simulink model "ElevatorPlant_Storage_A"  (R2015b)
settings: Solver=VariableStepAuto  StartTime=0.0  StopTime=10.0  RelTol=1e-3
(part 2 of 8)

== stateflow chart ElevatorPlant_Storage_A/Elevator Plant_storage ==
  state Init_procedure
    state BLK_Init
      %BLK(LPS0)
      %BLK(LPD1)
      %BLK(LPS1)
      %BLK(LPD2)
      %BLK(LPS2)
      %BLK(LPD3)
    state Closing_all_doors
      state Closing0
        state Reset
          state Reset_0
            en:
            LPS0=false;
            BUTTON_CAR(1)=false;
            BUTTON_UP(1)=false;
          state Reset_1
            en:
            LPS1=false;
            LPD1=false;
            BUTTON_CAR(2)=false;
            BUTTON_UP(2)=false;
            BUTTON_DOWN(2)=false;
          state Reset_2
            en:
            LPS2=false;
            LPD2=false;
            BUTTON_CAR(3)=false;
            BUTTON_UP(3)=false;
            BUTTON_DOWN(3)=false;
          state Reset_3
            en:
            LPD3=false;
            BUTTON_CAR(4)=false;
            BUTTON_DOWN(4)=false;
          (default) -> (junction 27093)
          (junction 27093) -> Init_procedure.Closing_all_doors.Closing0.Reset.Reset_0 [order 1] : [FLOOR==0]
          Init_procedure.Closing_all_doors.Closing0.Reset.Reset_0 -> (junction 27101)
          (junction 27093) -> (junction 27095) [order 2]
          (junction 27101) -> (junction 27103)
          (junction 27095) -> Init_procedure.Closing_all_doors.Closing0.Reset.Reset_1 [order 1] : [FLOOR==1]
          Init_procedure.Closing_all_doors.Closing0.Reset.Reset_1 -> (junction 27103)
          (junction 27095) -> (junction 27097) [order 2]
          (junction 27103) -> (junction 27104)
          (junction 27097) -> Init_procedure.Closing_all_doors.Closing0.Reset.Reset_2 [order 1] : [FLOOR==2]
          Init_procedure.Closing_all_doors.Closing0.Reset.Reset_2 -> (junction 27104)
          (junction 27097) -> (junction 27099) [order 2]
          (junction 27104) -> (junction 27109)
          (junction 27099) -> Init_procedure.Closing_all_doors.Closing0.Reset.Reset_3 [order 1] : [FLOOR==3]
          Init_procedure.Closing_all_doors.Closing0.Reset.Reset_3 -> (junction 27109)
          (junction 27099) -> (junction 27114) [order 2]
          (junction 27109) -> (junction 27115)
          (junction 27115) -> (junction 27114)
        state Timer_close
          state Set_tmr
            en: Q_cl=true;
          state Set
            en:PT_cl=5;
            IN_cl=true;
          state Counting
            en:ET_cl = ET_cl + 1;
            Q_cl=false;
          (junction 11293) -> Init_procedure.Closing_all_doors.Closing0.Timer_close.Set_tmr [order 1] : [ET_cl==PT_cl]
          Init_procedure.Closing_all_doors.Closing0.Timer_close.Set_tmr -> (junction 11294)
          (default) -> Init_procedure.Closing_all_doors.Closing0.Timer_close.Set
          Init_procedure.Closing_all_doors.Closing0.Timer_close.Counting -> (junction 11293)
          (junction 11293) -> (junction 11294) [order 2]
          Init_procedure.Closing_all_doors.Closing0.Timer_close.Set -> (junction 11295)
          (junction 11295) -> Init_procedure.Closing_all_doors.Closing0.Timer_close.Counting [order 1] : [ET_cl<PT_cl]
          (junction 11295) -> (junction 11294) [order 2]
        state Closing
          en: CP0=Q_cl;
        state Button_detection
          state Save_energy
            en:
            LL=not(Q_LL);
          state Timer_LL
            state Set_tmr
              en:
              Q_LL=true;
            state Counting
              en:
              ET_LL= ET_LL + 1;
              Q_LL=false;
            state Set
              en:
              IN_LL=true;
              PT_LL=10;
            (junction 66372) -> Init_procedure.Closing_all_doors.Closing0.Button_detection.Timer_LL.Set_tmr [order 1] : [ET_LL==PT_LL]
            Init_procedure.Closing_all_doors.Closing0.Button_detection.Timer_LL.Set_tmr -> (junction 66373)
            Init_procedure.Closing_all_doors.Closing0.Button_detection.Timer_LL.Counting -> (junction 66372)
            (junction 66372) -> (junction 66373) [order 2]
            (default) -> Init_procedure.Closing_all_doors.Closing0.Button_detection.Timer_LL.Set
            Init_procedure.Closing_all_doors.Closing0.Button_detection.Timer_LL.Set -> (junction 66374)
            (junction 66374) -> Init_procedure.Closing_all_doors.Closing0.Button_detection.Timer_LL.Counting [order 1] : [ET_LL<PT_LL]
            (junction 66374) -> (junction 66373) [order 2]
          state BUTTON_DOWN
            state Button_DOWN_1
              en:
              BUTTON_DOWN(2)=true;
              BUT_TEMP=1;
              LPD1=true;
              PUSHED=true;
              UPDATE=false;
              IN_LL=false; ET_LL=0;
            state First_but_1
              en:
              BUT_1=BUT_TEMP;
              FIRST_BUT=false;
            state Button_DOWN_2
              en:
              BUTTON_DOWN(3)=true;
              BUT_TEMP=2;
              LPD2=true;
              PUSHED=true;
              UPDATE=false;
              IN_LL=false; ET_LL=0;
            state First_but_2
              en:
              BUT_1=BUT_TEMP;
              FIRST_BUT=false;
            state Button_DOWN_3
              en:
              BUTTON_DOWN(4)=true;
              BUT_TEMP=3;
              LPD3=true;
              PUSHED=true;
              UPDATE=false;
              IN_LL=false; ET_LL=0;
            state First_but_3
              en:
              BUT_1=BUT_TEMP;
              FIRST_BUT=false;
            (default) -> (junction 66387)
            (junction 66387) -> Init_procedure.Closing_all_doors.Closing0.Button_detection.BUTTON_DOWN.Button_DOWN_1 [order 1] : [PD1]
            Init_procedure.Closing_all_doors.Closing0.Button_detection.BUTTON_DOWN.Button_DOWN_1 -> (junction 66388)
            (junction 66388) -> Init_procedure.Closing_all_doors.Closing0.Button_detection.BUTTON_DOWN.First_but_1 [order 1] : [FIRST_BUT && not(RPC1)]
            Init_procedure.Closing_all_doors.Closing0.Button_detection.BUTTON_DOWN.First_but_1 -> (junction 66389)
            (junction 66387) -> (junction 66390) [order 2]
            (junction 66388) -> (junction 66391) [order 2]
            (junction 66389) -> (junction 66392)
            (junction 66391) -> (junction 66390)
            (junction 66392) -> (junction 66391)
            (junction 66390) -> (junction 66393)
            (junction 66393) -> Init_procedure.Closing_all_doors.Closing0.Button_detection.BUTTON_DOWN.Button_DOWN_2 [order 1] : [PD2]
            Init_procedure.Closing_all_doors.Closing0.Button_detection.BUTTON_DOWN.Button_DOWN_2 -> (junction 66394)
            (junction 66394) -> Init_procedure.Closing_all_doors.Closing0.Button_detection.BUTTON_DOWN.First_but_2 [order 1] : [FIRST_BUT && not(RPC2)]
            Init_procedure.Closing_all_doors.Closing0.Button_detection.BUTTON_DOWN.First_but_2 -> (junction 66395)
            (junction 66393) -> (junction 66396) [order 2]
            (junction 66394) -> (junction 66397) [order 2]
            (junction 66395) -> (junction 66398)
            (junction 66397) -> (junction 66396)
            (junction 66398) -> (junction 66397)
            (junction 66396) -> (junction 66399)
            (junction 66399) -> Init_procedure.Closing_all_doors.Closing0.Button_detection.BUTTON_DOWN.Button_DOWN_3 [order 1] : [PD3]
            Init_procedure.Closing_all_doors.Closing0.Button_detection.BUTTON_DOWN.Button_DOWN_3 -> (junction 66400)
            (junction 66400) -> Init_procedure.Closing_all_doors.Closing0.Button_detection.BUTTON_DOWN.First_but_3 [order 1] : [FIRST_BUT && not(RPC3)]
            Init_procedure.Closing_all_doors.Closing0.Button_detection.BUTTON_DOWN.First_but_3 -> (junction 66401)
            (junction 66399) -> (junction 66402) [order 2]
            (junction 66400) -> (junction 66403) [order 2]
            (junction 66401) -> (junction 66404)
            (junction 66403) -> (junction 66402)
            (junction 66404) -> (junction 66403)
          state BUTTON_CAR
            state Button_CAR_0
              en:
              BUTTON_CAR(1)=true;
              BUT_TEMP=0;
              LPC0=true;
              PUSHED=true;
              UPDATE=false;
              IN_LL=false; ET_LL=0;
            state First_but_0
              en:
              BUT_1=BUT_TEMP;
              FIRST_BUT=false;
            state Button_CAR_1
              en:
              BUTTON_CAR(2)=true;
              BUT_TEMP=1;
              LPC1=true;
              PUSHED=true;
              UPDATE=false;
              IN_LL=false; ET_LL=0;
            state First_but_1
              en:
              BUT_1=BUT_TEMP;
              FIRST_BUT=false;
            state Button_CAR_2
              en:
              BUTTON_CAR(3)=true;
              BUT_TEMP=2;
              LPC2=true;
              PUSHED=true;
              UPDATE=false;
              IN_LL=false; ET_LL=0;
            state First_but_2
              en:
              BUT_1=BUT_TEMP;
              FIRST_BUT=false;
            state Button_CAR_3
              en:
              BUTTON_CAR(4)=true;
              BUT_TEMP=3;
              LPC3=true;
              PUSHED=true;
              UPDATE=false;
              IN_LL=false; ET_LL=0;
            state First_but_3
              en:
              BUT_1=BUT_TEMP;
              FIRST_BUT=false;
            (default) -> (junction 66442)
            (junction 66442) -> Init_procedure.Closing_all_doors.Closing0.Button_detection.BUTTON_CAR.Button_CAR_0 [order 1] : [P0]
            Init_procedure.Closing_all_doors.Closing0.Button_detection.BUTTON_CAR.Button_CAR_0 -> (junction 66443)
            (junction 66443) -> Init_procedure.Closing_all_doors.Closing0.Button_detection.BUTTON_CAR.First_but_0 [order 1] : [FIRST_BUT && not(RPC0)]
            Init_procedure.Closing_all_doors.Closing0.Button_detection.BUTTON_CAR.First_but_0 -> (junction 66444)
            (junction 66442) -> (junction 66445) [order 2]
            (junction 66443) -> (junction 66446) [order 2]
            (junction 66444) -> (junction 66447)
            (junction 66446) -> (junction 66445)
            (junction 66447) -> (junction 66446)
            (junction 66445) -> (junction 66450)
            Init_procedure.Closing_all_doors.Closing0.Button_detection.BUTTON_CAR.Button_CAR_1 -> (junction 66448)
            (junction 66448) -> Init_procedure.Closing_all_doors.Closing0.Button_detection.BUTTON_CAR.First_but_1 [order 1] : [FIRST_BUT && not(RPC1)]
            Init_procedure.Closing_all_doors.Closing0.Button_detection.BUTTON_CAR.First_but_1 -> (junction 66449)
            (junction 66448) -> (junction 66452) [order 2]
            (junction 66449) -> (junction 66453)
            (junction 66450) -> Init_procedure.Closing_all_doors.Closing0.Button_detection.BUTTON_CAR.Button_CAR_1 [order 1] : [P1]
            (junction 66450) -> (junction 66451) [order 2]
            (junction 66452) -> (junction 66451)
            (junction 66453) -> (junction 66452)
            (junction 66451) -> (junction 66454)
            (junction 66454) -> Init_procedure.Closing_all_doors.Closing0.Button_detection.BUTTON_CAR.Button_CAR_2 [order 1] : [P2]
            Init_procedure.Closing_all_doors.Closing0.Button_detection.BUTTON_CAR.Button_CAR_2 -> (junction 66455)
            (junction 66455) -> Init_procedure.Closing_all_doors.Closing0.Button_detection.BUTTON_CAR.First_but_2 [order 1] : [FIRST_BUT && not(RPC2)]
            Init_procedure.Closing_all_doors.Closing0.Button_detection.BUTTON_CAR.First_but_2 -> (junction 66456)
            (junction 66454) -> (junction 66457) [order 2]
            (junction 66455) -> (junction 66458) [order 2]
            (junction 66456) -> (junction 66459)
            (junction 66458) -> (junction 66457)
            (junction 66459) -> (junction 66458)
            (junction 66457) -> (junction 66460)
            (junction 66460) -> Init_procedure.Closing_all_doors.Closing0.Button_detection.BUTTON_CAR.Button_CAR_3 [order 1] : [P3]
            Init_procedure.Closing_all_doors.Closing0.Button_detection.BUTTON_CAR.Button_CAR_3 -> (junction 66461)
            (junction 66461) -> Init_procedure.Closing_all_doors.Closing0.Button_detection.BUTTON_CAR.First_but_3 [order 1] : [FIRST_BUT && not(RPC3)]
            Init_procedure.Closing_all_doors.Closing0.Button_detection.BUTTON_CAR.First_but_3 -> (junction 66462)
            (junction 66460) -> (junction 66463) [order 2]
            (junction 66461) -> (junction 66464) [order 2]
            (junction 66462) -> (junction 66465)
            (junction 66464) -> (junction 66463)
            (junction 66465) -> (junction 66464)
          state BUTTON_UP
            state Button_UP_0
              en:
              BUTTON_UP(1)=true;
              BUT_TEMP=0;
              LPS0=true;
              PUSHED=true;
              UPDATE=false;
              IN_LL=false; ET_LL=0;
            state First_but_0
              en:
              BUT_1=BUT_TEMP;
              FIRST_BUT=false;
            state Button_UP_1
              en:
              BUTTON_UP(2)=true;
              BUT_TEMP=1;
              LPS1=true;
              PUSHED=true;
              UPDATE=false;
              IN_LL=false; ET_LL=0;
            state First_but_1
              en:
              BUT_1=BUT_TEMP;
              FIRST_BUT=false;
            state Button_UP_2
              en:
              BUTTON_UP(3)=true;
              BUT_TEMP=2;
              LPS2=true;
              PUSHED=true;
              UPDATE=false;
              IN_LL=false; ET_LL=0;
            state First_but_2
              en:
              BUT_1=BUT_TEMP;
              FIRST_BUT=false;
            (junction 66515) -> Init_procedure.Closing_all_doors.Closing0.Button_detection.BUTTON_UP.Button_UP_0 [order 1] : [PS0]
            Init_procedure.Closing_all_doors.Closing0.Button_detection.BUTTON_UP.Button_UP_0 -> (junction 66516)
            (junction 66516) -> Init_procedure.Closing_all_doors.Closing0.Button_detection.BUTTON_UP.First_but_0 [order 1] : [FIRST_BUT && not(RPC0)]
            Init_procedure.Closing_all_doors.Closing0.Button_detection.BUTTON_UP.First_but_0 -> (junction 66517)
            (default) -> (junction 66515)
            (junction 66515) -> (junction 66520) [order 2]
            (junction 66516) -> (junction 66518) [order 2]
            (junction 66517) -> (junction 66519)
            (junction 66519) -> (junction 66518)
            (junction 66518) -> (junction 66520)
            (junction 66520) -> (junction 66521)
            (junction 66521) -> Init_procedure.Closing_all_doors.Closing0.Button_detection.BUTTON_UP.Button_UP_1 [order 1] : [PS1]
            Init_procedure.Closing_all_doors.Closing0.Button_detection.BUTTON_UP.Button_UP_1 -> (junction 66522)
            (junction 66522) -> Init_procedure.Closing_all_doors.Closing0.Button_detection.BUTTON_UP.First_but_1 [order 1] : [FIRST_BUT && not(RPC1)]
            Init_procedure.Closing_all_doors.Closing0.Button_detection.BUTTON_UP.First_but_1 -> (junction 66523)
            (junction 66521) -> (junction 66524) [order 2]
            (junction 66522) -> (junction 66525) [order 2]
            (junction 66523) -> (junction 66526)
            (junction 66525) -> (junction 66524)
            (junction 66526) -> (junction 66525)
            (junction 66524) -> (junction 66528)
            Init_procedure.Closing_all_doors.Closing0.Button_detection.BUTTON_UP.First_but_2 -> (junction 66527)
            (junction 66527) -> (junction 66532)
            (junction 66528) -> Init_procedure.Closing_all_doors.Closing0.Button_detection.BUTTON_UP.Button_UP_2 [order 1] : [PS2]
            Init_procedure.Closing_all_doors.Closing0.Button_detection.BUTTON_UP.Button_UP_2 -> (junction 66529)
            (junction 66529) -> Init_procedure.Closing_all_doors.Closing0.Button_detection.BUTTON_UP.First_but_2 [order 1] : [FIRST_BUT && not(RPC2)]
            (junction 66528) -> (junction 66530) [order 2]
            (junction 66529) -> (junction 66531) [order 2]
            (junction 66531) -> (junction 66530)
            (junction 66532) -> (junction 66531)
          state Max_Min_assignment
            state Min_but
              en:
              BUTTON=MIN_BUT;
            state Max_but
              en:
              BUTTON=MAX_BUT;
            state First_but
              en:
              BUTTON=BUT_1;
            state Max_but1
              en:
              MAX_BUT=2;
            state Max_but2
              en:
              MAX_BUT=1;
            state Max_but3
              en:
              MAX_BUT=0;
            state Min_but1
              en:
              MIN_BUT=1;
            state Min_but2
              en:
              MIN_BUT=2;
            state Min_but3
              en:
              MIN_BUT=3;
            state MAX
              en:
              MAX_BUT=BUT_TEMP;
            state MIN
              en:
              MIN_BUT=BUT_TEMP;
            state Updating_button_0
              en:
              BUTTON=MAX_BUT;
            state Updating_button_1
              en:
              BUTTON=MIN_BUT;
            (junction 66570) -> Init_procedure.Closing_all_doors.Closing0.Button_detection.Max_Min_assignment.Min_but [order 1] : [(MAX_BUT-FLOOR)>(FLOOR-MIN_BUT)]
            Init_procedure.Closing_all_doors.Closing0.Button_detection.Max_Min_assignment.Min_but -> (junction 66571)
            (junction 66572) -> (junction 66570) [order 1] : [not(FLAG_STOP) && MOTION==2 && FLAG==3]
            (default) -> (junction 66572)
            (junction 66570) -> (junction 66573) [order 2]
            (junction 66571) -> (junction 66574)
            (junction 66572) -> (junction 66575) [order 2]
            (junction 66573) -> Init_procedure.Closing_all_doors.Closing0.Button_detection.Max_Min_assignment.Max_but [order 1] : [(MAX_BUT-FLOOR)<(FLOOR-MIN_BUT)]
            Init_procedure.Closing_all_doors.Closing0.Button_detection.Max_Min_assignment.Max_but -> (junction 66574)
            (junction 66573) -> Init_procedure.Closing_all_doors.Closing0.Button_detection.Max_Min_assignment.First_but [order 2]
            (junction 66574) -> (junction 66577)
            Init_procedure.Closing_all_doors.Closing0.Button_detection.Max_Min_assignment.First_but -> (junction 66576)
            (junction 66576) -> (junction 66575)
            (junction 66577) -> (junction 66576)
            (junction 66575) -> (junction 66578)
            (junction 66579) -> (junction 66580) [order 1] : [MOTION==0]
                | {MOTION=1;
                | UPDATE=true;}
            (junction 66580) -> Init_procedure.Closing_all_doors.Closing0.Button_detection.Max_Min_assignment.Max_but1 [order 1] : [BUTTON_UP(2)]
            Init_procedure.Closing_all_doors.Closing0.Button_detection.Max_Min_assignment.Max_but1 -> (junction 66581)
            (junction 66578) -> (junction 66579) [order 1] : [BUTTON==FLOOR && EXTEND]
                | {EXTEND=false;}
            (junction 66578) -> (junction 66592) [order 2]
            (junction 66579) -> (junction 66584) [order 2]
            (junction 66580) -> (junction 66582) [order 2]
            (junction 66581) -> (junction 66583)
            (junction 66582) -> Init_procedure.Closing_all_doors.Closing0.Button_detection.Max_Min_assignment.Max_but2 [order 1] : [BUTTON_UP(1)]
            Init_procedure.Closing_all_doors.Closing0.Button_detection.Max_Min_assignment.Max_but2 -> (junction 66583)
            (junction 66582) -> Init_procedure.Closing_all_doors.Closing0.Button_detection.Max_Min_assignment.Max_but3 [order 2]
            (junction 66583) -> (junction 66586)
            Init_procedure.Closing_all_doors.Closing0.Button_detection.Max_Min_assignment.Max_but3 -> (junction 66585)
            (junction 66585) -> (junction 66584)
            (junction 66586) -> (junction 66585)
            (junction 66584) -> (junction 66587)
            (junction 66587) -> (junction 66588) [order 1] : [MOTION==1]
                | {MOTION=0;
                | UPDATE=true;}
            (junction 66588) -> Init_procedure.Closing_all_doors.Closing0.Button_detection.Max_Min_assignment.Min_but1 [order 1] : [BUTTON_DOWN(1)]
            Init_procedure.Closing_all_doors.Closing0.Button_detection.Max_Min_assignment.Min_but1 -> (junction 66589)
            (junction 66587) -> (junction 66593) [order 2]
            (junction 66588) -> (junction 66590) [order 2]
            (junction 66589) -> (junction 66591)
            (junction 66590) -> Init_procedure.Closing_all_doors.Closing0.Button_detection.Max_Min_assignment.Min_but2 [order 1] : [BUTTON_DOWN(2)]
            Init_procedure.Closing_all_doors.Closing0.Button_detection.Max_Min_assignment.Min_but2 -> (junction 66591)
            (junction 66590) -> Init_procedure.Closing_all_doors.Closing0.Button_detection.Max_Min_assignment.Min_but3 [order 2]
            (junction 66591) -> (junction 66595)
            Init_procedure.Closing_all_doors.Closing0.Button_detection.Max_Min_assignment.Min_but3 -> (junction 66594)
            (junction 66593) -> (junction 66592)
            (junction 66594) -> (junction 66593)
            (junction 66595) -> (junction 66594)
            (junction 66592) -> (junction 66597)
            Init_procedure.Closing_all_doors.Closing0.Button_detection.Max_Min_assignment.MAX -> (junction 66596)
            (junction 66597) -> (junction 66598) [order 1] : [PUSHED]
            (junction 66598) -> (junction 66599) [order 1] : [not(BUT_TEMP==FLOOR) || not(MOTION==2)]
            (junction 66599) -> Init_procedure.Closing_all_doors.Closing0.Button_detection.Max_Min_assignment.MAX [order 1] : [MAX_BUT<BUT_TEMP && not(UPDATE)]
            (junction 66596) -> (junction 66601)
            (junction 66597) -> (junction 66611) [order 2]
            (junction 66598) -> (junction 66604) [order 2]
            (junction 66599) -> (junction 66600) [order 2]
            (junction 66601) -> (junction 66600)
            (junction 66600) -> (junction 66602)
            (junction 66602) -> Init_procedure.Closing_all_doors.Closing0.Button_detection.Max_Min_assignment.MIN [order 1] : [MIN_BUT>BUT_TEMP && not(UPDATE)]
            Init_procedure.Closing_all_doors.Closing0.Button_detection.Max_Min_assignment.MIN -> (junction 66603)
            (junction 66602) -> (junction 66605) [order 2]
            (junction 66603) -> (junction 66606)
            (junction 66605) -> (junction 66604)
            (junction 66606) -> (junction 66605)
            (junction 66604) -> (junction 66607)
            (junction 66607) -> Init_procedure.Closing_all_doors.Closing0.Button_detection.Max_Min_assignment.Updating_button_0 [order 1] : [MOTION==0]
            Init_procedure.Closing_all_doors.Closing0.Button_detection.Max_Min_assignment.Updating_button_0 -> (junction 66608)
            (junction 66607) -> (junction 66609) [order 2]
            (junction 66608) -> (junction 66610)
            (junction 66609) -> Init_procedure.Closing_all_doors.Closing0.Button_detection.Max_Min_assignment.Updating_button_1 [order 1] : [MOTION==1]
            Init_procedure.Closing_all_doors.Closing0.Button_detection.Max_Min_assignment.Updating_button_1 -> (junction 66610)
            (junction 66609) -> (junction 66612) [order 2]
            (junction 66610) -> (junction 66613)
            (junction 66612) -> (junction 66611)
            (junction 66613) -> (junction 66612)
          state GoTo_PositionControl
            en:
            BUTTON=BUT_TEMP;
            FLAG=2;
          state Emergency
            en:
            FLAG_EMG=true;
            FLAG=4;
          state Timer_EME
            state Set_tmr
              en:
              Q_EME=true;
            state Counting
              en:
              ET_EME= ET_EME + 1;
              Q_EME=false;
            state Set
              en:
              IN_EME=true;
              PT_EME=3;
            (junction 66703) -> Init_procedure.Closing_all_doors.Closing0.Button_detection.Timer_EME.Set_tmr [order 1] : [ET_EME==PT_EME]
            Init_procedure.Closing_all_doors.Closing0.Button_detection.Timer_EME.Set_tmr -> (junction 66704)
            Init_procedure.Closing_all_doors.Closing0.Button_detection.Timer_EME.Counting -> (junction 66703)
            (junction 66703) -> (junction 66704) [order 2]
            (default) -> Init_procedure.Closing_all_doors.Closing0.Button_detection.Timer_EME.Set
            Init_procedure.Closing_all_doors.Closing0.Button_detection.Timer_EME.Set -> (junction 66705)
            (junction 66705) -> Init_procedure.Closing_all_doors.Closing0.Button_detection.Timer_EME.Counting [order 1] : [ET_EME<PT_EME]
            (junction 66705) -> (junction 66704) [order 2]
          state Not_Emergency
            en:
            IN_EME=false;
            ET_EME=0;
          state SwitchingOFF_LEDs
            en:
            LPD3=false;
            LPD2=false;
            LPS2=false;
            LPD1=false;
            LPS1=false;
            LPS0=false;
          (default) -> (junction 66304)
          (junction 66304) -> (junction 66305) [order 1] : [FLAG==1 && not(PUSHED)]
              | {BUTTON=FLOOR;
              | BUT_TEMP=BUTTON;
              | BUT_1=FLOOR;}
          (junction 66305) -> Init_procedure.Closing_all_doors.Closing0.Button_detection.Timer_LL [order 1] : [not(FLAG_STOP)]
          Init_procedure.Closing_all_doors.Closing0.Button_detection.Save_energy -> (junction 66306)
          Init_procedure.Closing_all_doors.Closing0.Button_detection.Timer_LL -> Init_procedure.Closing_all_doors.Closing0.Button_detection.Save_energy
          (junction 66305) -> (junction 66308) [order 2]
          (junction 66304) -> (junction 66307) [order 2]
          (junction 66306) -> (junction 66309)
          (junction 66308) -> (junction 66307)
          (junction 66309) -> (junction 66308)
          (junction 66307) -> Init_procedure.Closing_all_doors.Closing0.Button_detection.BUTTON_CAR
          Init_procedure.Closing_all_doors.Closing0.Button_detection.BUTTON_UP -> Init_procedure.Closing_all_doors.Closing0.Button_detection.BUTTON_DOWN
          Init_procedure.Closing_all_doors.Closing0.Button_detection.BUTTON_DOWN -> Init_procedure.Closing_all_doors.Closing0.Button_detection.Max_Min_assignment
          Init_procedure.Closing_all_doors.Closing0.Button_detection.Max_Min_assignment -> (junction 66310)
          Init_procedure.Closing_all_doors.Closing0.Button_detection.BUTTON_CAR -> Init_procedure.Closing_all_doors.Closing0.Button_detection.BUTTON_UP
          (junction 66310) -> (junction 66312)
          (junction 66312) -> (junction 66311)
          (junction 66311) -> (junction 66314)
          Init_procedure.Closing_all_doors.Closing0.Button_detection.GoTo_PositionControl -> (junction 66313)
          (junction 66314) -> (junction 66315) [order 1] : [FLAG==1]
          (junction 66315) -> Init_procedure.Closing_all_doors.Closing0.Button_detection.GoTo_PositionControl [order 1] : [PUSHED]
          (junction 66313) -> (junction 66317)
          (junction 66314) -> (junction 66325) [order 2]
          (junction 66315) -> (junction 66316) [order 2]
          (junction 66317) -> (junction 66316)
          (junction 66316) -> (junction 66319)
          Init_procedure.Closing_all_doors.Closing0.Button_detection.Emergency -> (junction 66318)
          (junction 66319) -> Init_procedure.Closing_all_doors.Closing0.Button_detection.Timer_EME [order 1] : [STOP]
              | {IN_LL=false; ET_LL=0;FLAG=1;}
          Init_procedure.Closing_all_doors.Closing0.Button_detection.Timer_EME -> (junction 66320)
          (junction 66320) -> Init_procedure.Closing_all_doors.Closing0.Button_detection.Emergency [order 1] : [Q_EME]
          (junction 66318) -> (junction 66322)
          (junction 66319) -> Init_procedure.Closing_all_doors.Closing0.Button_detection.Not_Emergency [order 2]
          (junction 66320) -> (junction 66321) [order 2]
          (junction 66322) -> (junction 66321)
          (junction 66321) -> (junction 66324)
          Init_procedure.Closing_all_doors.Closing0.Button_detection.Not_Emergency -> (junction 66324)
          Init_procedure.Closing_all_doors.Closing0.Button_detection.SwitchingOFF_LEDs -> (junction 66323)
          (junction 66324) -> Init_procedure.Closing_all_doors.Closing0.Button_detection.SwitchingOFF_LEDs [order 1] : [FLAG_STOP && FLAG==2]
          (junction 66323) -> (junction 66327)
          (junction 66324) -> (junction 66326) [order 2]
          (junction 66326) -> (junction 66325)
          (junction 66327) -> (junction 66326)
        state Extending
          en:
          EXTEND=true;
        state Stop_Closing
          en:
          CP0=false;
          FLAG_OD=false;
          OBS=false;
          ET_cl=0;
          IN_cl=false;
        state GoTo_PositionControl
          en: FLAG=2;
        state GoTo_BUttonDetection
          en:
          MOTION=2;
          MAX_BUT=0;
          MIN_BUT=3;
          PUSHED=false;
          FIRST_BUT=true;
          FLAG=1;
          UPDATE=false;
        state Closing1
          en:CP0=true;
        state Stop_Closing1
          en:CP0=false;
        Init_procedure.Closing_all_doors.Closing0.Reset -> Init_procedure.Closing_all_doors.Closing0.Timer_close
        (default) -> (junction 11265)
        (junction 11265) -> Init_procedure.Closing_all_doors.Closing0.Reset [order 1] : [not(FLAG==0) && not(FLAG==4)]
        Init_procedure.Closing_all_doors.Closing0.Timer_close -> (junction 11264)
        (junction 11264) -> Init_procedure.Closing_all_doors.Closing0.Closing [order 1] : [not(PC0)]
        Init_procedure.Closing_all_doors.Closing0.Button_detection -> (junction 27077)
        Init_procedure.Closing_all_doors.Closing0.Closing -> Init_procedure.Closing_all_doors.Closing0.Button_detection
        (junction 11265) -> (junction 11267) [order 2]
        (junction 11264) -> (junction 65270) [order 2]
        (junction 27077) -> (junction 27082)
        (junction 65270) -> Init_procedure.Closing_all_doors.Closing0.Extending [order 1] : [BUTTON==FLOOR]
        (junction 65270) -> (junction 65274) [order 2]
        Init_procedure.Closing_all_doors.Closing0.Extending -> (junction 65278)
        (junction 65278) -> (junction 65274)
        (junction 65274) -> Init_procedure.Closing_all_doors.Closing0.Stop_Closing
        Init_procedure.Closing_all_doors.Closing0.Stop_Closing -> (junction 11266)
        (junction 11266) -> Init_procedure.Closing_all_doors.Closing0.GoTo_PositionControl [order 2]
        (junction 11266) -> Init_procedure.Closing_all_doors.Closing0.GoTo_BUttonDetection [order 1] : [not(BUTTON_CAR(1) || BUTTON_CAR(2) || BUTTON_CAR(3) || BUTTON_CAR(4) || BUTTON_UP(1) || BUTTON_UP(2) || BUTTON_UP(3) || BUTTON_DOWN(2) || BUTTON_DOWN(3) || BUTTON_DOWN(4))]
        Init_procedure.Closing_all_doors.Closing0.GoTo_PositionControl -> (junction 27079)
        Init_procedure.Closing_all_doors.Closing0.GoTo_BUttonDetection -> (junction 27079)
        (junction 27079) -> (junction 27082)
        (junction 27082) -> (junction 27087)
        (junction 27087) -> (junction 27090)
        (junction 11267) -> Init_procedure.Closing_all_doors.Closing0.Closing1 [order 1] : [not(PC0)]
        Init_procedure.Closing_all_doors.Closing0.Closing1 -> (junction 27090)
        (junction 11267) -> Init_procedure.Closing_all_doors.Closing0.Stop_Closing1 [order 2]
        Init_procedure.Closing_all_doors.Closing0.Stop_Closing1 -> (junction 27090)
      state Closing1
        state Reset
          state Reset_0
            en:
            LPS0=false;
            BUTTON_CAR(1)=false;
            BUTTON_UP(1)=false;
          state Reset_1
            en:
            LPS1=false;
            LPD1=false;
            BUTTON_CAR(2)=false;
            BUTTON_UP(2)=false;
            BUTTON_DOWN(2)=false;
          state Reset_2
            en:
            LPS2=false;
            LPD2=false;
            BUTTON_CAR(3)=false;
            BUTTON_UP(3)=false;
            BUTTON_DOWN(3)=false;
          state Reset_3
            en:
            LPD3=false;
            BUTTON_CAR(4)=false;
            BUTTON_DOWN(4)=false;
          (default) -> (junction 65322)
          (junction 65322) -> Init_procedure.Closing_all_doors.Closing1.Reset.Reset_0 [order 1] : [FLOOR==0]
          Init_procedure.Closing_all_doors.Closing1.Reset.Reset_0 -> (junction 65323)
          (junction 65322) -> (junction 65324) [order 2]
          (junction 65323) -> (junction 65325)
          (junction 65324) -> Init_procedure.Closing_all_doors.Closing1.Reset.Reset_1 [order 1] : [FLOOR==1]
          Init_procedure.Closing_all_doors.Closing1.Reset.Reset_1 -> (junction 65325)
          (junction 65324) -> (junction 65326) [order 2]
          (junction 65325) -> (junction 65327)
          (junction 65326) -> Init_procedure.Closing_all_doors.Closing1.Reset.Reset_2 [order 1] : [FLOOR==2]
          Init_procedure.Closing_all_doors.Closing1.Reset.Reset_2 -> (junction 65327)
          (junction 65326) -> (junction 65328) [order 2]
          (junction 65327) -> (junction 65329)
          (junction 65328) -> Init_procedure.Closing_all_doors.Closing1.Reset.Reset_3 [order 1] : [FLOOR==3]
          Init_procedure.Closing_all_doors.Closing1.Reset.Reset_3 -> (junction 65329)
          (junction 65328) -> (junction 65330) [order 2]
          (junction 65329) -> (junction 65331)
          (junction 65331) -> (junction 65330)
        state Timer_close
          state Set_tmr
            en: Q_cl=true;
          state Set
            en:PT_cl=5;
            IN_cl=true;
          state Counting
            en:ET_cl = ET_cl + 1;
            Q_cl=false;
          (junction 65355) -> Init_procedure.Closing_all_doors.Closing1.Timer_close.Set_tmr [order 1] : [ET_cl==PT_cl]
          Init_procedure.Closing_all_doors.Closing1.Timer_close.Set_tmr -> (junction 65356)
          (default) -> Init_procedure.Closing_all_doors.Closing1.Timer_close.Set
          Init_procedure.Closing_all_doors.Closing1.Timer_close.Counting -> (junction 65355)
          (junction 65355) -> (junction 65356) [order 2]
          Init_procedure.Closing_all_doors.Closing1.Timer_close.Set -> (junction 65357)
          (junction 65357) -> Init_procedure.Closing_all_doors.Closing1.Timer_close.Counting [order 1] : [ET_cl<PT_cl]
          (junction 65357) -> (junction 65356) [order 2]
        state Closing
          en: CP1=Q_cl;
        state Button_detection
          state Save_energy
            en:
            LL=not(Q_LL);
          state Timer_LL
            state Set_tmr
              en:
              Q_LL=true;
            state Counting
              en:
              ET_LL= ET_LL + 1;
              Q_LL=false;
            state Set
              en:
              IN_LL=true;
              PT_LL=10;
            (junction 66788) -> Init_procedure.Closing_all_doors.Closing1.Button_detection.Timer_LL.Set_tmr [order 1] : [ET_LL==PT_LL]
            Init_procedure.Closing_all_doors.Closing1.Button_detection.Timer_LL.Set_tmr -> (junction 66789)
            Init_procedure.Closing_all_doors.Closing1.Button_detection.Timer_LL.Counting -> (junction 66788)
            (junction 66788) -> (junction 66789) [order 2]
            (default) -> Init_procedure.Closing_all_doors.Closing1.Button_detection.Timer_LL.Set
            Init_procedure.Closing_all_doors.Closing1.Button_detection.Timer_LL.Set -> (junction 66790)
            (junction 66790) -> Init_procedure.Closing_all_doors.Closing1.Button_detection.Timer_LL.Counting [order 1] : [ET_LL<PT_LL]
            (junction 66790) -> (junction 66789) [order 2]
          state BUTTON_DOWN
            state Button_DOWN_1
              en:
              BUTTON_DOWN(2)=true;
              BUT_TEMP=1;
              LPD1=true;
              PUSHED=true;
              UPDATE=false;
              IN_LL=false; ET_LL=0;
            state First_but_1
              en:
              BUT_1=BUT_TEMP;
              FIRST_BUT=false;
            state Button_DOWN_2
              en:
              BUTTON_DOWN(3)=true;
              BUT_TEMP=2;
              LPD2=true;
              PUSHED=true;
              UPDATE=false;
              IN_LL=false; ET_LL=0;
            state First_but_2
              en:
              BUT_1=BUT_TEMP;
              FIRST_BUT=false;
            state Button_DOWN_3
              en:
              BUTTON_DOWN(4)=true;
              BUT_TEMP=3;
              LPD3=true;
              PUSHED=true;
              UPDATE=false;
              IN_LL=false; ET_LL=0;
            state First_but_3
              en:
              BUT_1=BUT_TEMP;
              FIRST_BUT=false;
            (default) -> (junction 66803)
            (junction 66803) -> Init_procedure.Closing_all_doors.Closing1.Button_detection.BUTTON_DOWN.Button_DOWN_1 [order 1] : [PD1]
            Init_procedure.Closing_all_doors.Closing1.Button_detection.BUTTON_DOWN.Button_DOWN_1 -> (junction 66804)
            (junction 66804) -> Init_procedure.Closing_all_doors.Closing1.Button_detection.BUTTON_DOWN.First_but_1 [order 1] : [FIRST_BUT && not(RPC1)]
            Init_procedure.Closing_all_doors.Closing1.Button_detection.BUTTON_DOWN.First_but_1 -> (junction 66805)
            (junction 66803) -> (junction 66806) [order 2]
            (junction 66804) -> (junction 66807) [order 2]
            (junction 66805) -> (junction 66808)
            (junction 66807) -> (junction 66806)
            (junction 66808) -> (junction 66807)
            (junction 66806) -> (junction 66809)
            (junction 66809) -> Init_procedure.Closing_all_doors.Closing1.Button_detection.BUTTON_DOWN.Button_DOWN_2 [order 1] : [PD2]
            Init_procedure.Closing_all_doors.Closing1.Button_detection.BUTTON_DOWN.Button_DOWN_2 -> (junction 66810)
            (junction 66810) -> Init_procedure.Closing_all_doors.Closing1.Button_detection.BUTTON_DOWN.First_but_2 [order 1] : [FIRST_BUT && not(RPC2)]
            Init_procedure.Closing_all_doors.Closing1.Button_detection.BUTTON_DOWN.First_but_2 -> (junction 66811)
            (junction 66809) -> (junction 66812) [order 2]
            (junction 66810) -> (junction 66813) [order 2]
            (junction 66811) -> (junction 66814)
            (junction 66813) -> (junction 66812)
            (junction 66814) -> (junction 66813)
            (junction 66812) -> (junction 66815)
            (junction 66815) -> Init_procedure.Closing_all_doors.Closing1.Button_detection.BUTTON_DOWN.Button_DOWN_3 [order 1] : [PD3]
            Init_procedure.Closing_all_doors.Closing1.Button_detection.BUTTON_DOWN.Button_DOWN_3 -> (junction 66816)
            (junction 66816) -> Init_procedure.Closing_all_doors.Closing1.Button_detection.BUTTON_DOWN.First_but_3 [order 1] : [FIRST_BUT && not(RPC3)]
            Init_procedure.Closing_all_doors.Closing1.Button_detection.BUTTON_DOWN.First_but_3 -> (junction 66817)
            (junction 66815) -> (junction 66818) [order 2]
            (junction 66816) -> (junction 66819) [order 2]
            (junction 66817) -> (junction 66820)
            (junction 66819) -> (junction 66818)
            (junction 66820) -> (junction 66819)
          state BUTTON_CAR
            state Button_CAR_0
              en:
              BUTTON_CAR(1)=true;
              BUT_TEMP=0;
              LPC0=true;
              PUSHED=true;
              UPDATE=false;
              IN_LL=false; ET_LL=0;
            state First_but_0
              en:
              BUT_1=BUT_TEMP;
              FIRST_BUT=false;
            state Button_CAR_1
              en:
              BUTTON_CAR(2)=true;
              BUT_TEMP=1;
              LPC1=true;
              PUSHED=true;
              UPDATE=false;
              IN_LL=false; ET_LL=0;
            state First_but_1
              en:
              BUT_1=BUT_TEMP;
              FIRST_BUT=false;
            state Button_CAR_2
              en:
              BUTTON_CAR(3)=true;
              BUT_TEMP=2;
              LPC2=true;
              PUSHED=true;
              UPDATE=false;
              IN_LL=false; ET_LL=0;
            state First_but_2
              en:
              BUT_1=BUT_TEMP;
              FIRST_BUT=false;
            state Button_CAR_3
              en:
              BUTTON_CAR(4)=true;
              BUT_TEMP=3;
              LPC3=true;
              PUSHED=true;
              UPDATE=false;
              IN_LL=false; ET_LL=0;
            state First_but_3
              en:
              BUT_1=BUT_TEMP;
              FIRST_BUT=false;
            (default) -> (junction 66858)
            (junction 66858) -> Init_procedure.Closing_all_doors.Closing1.Button_detection.BUTTON_CAR.Button_CAR_0 [order 1] : [P0]
            Init_procedure.Closing_all_doors.Closing1.Button_detection.BUTTON_CAR.Button_CAR_0 -> (junction 66859)
            (junction 66859) -> Init_procedure.Closing_all_doors.Closing1.Button_detection.BUTTON_CAR.First_but_0 [order 1] : [FIRST_BUT && not(RPC0)]
            Init_procedure.Closing_all_doors.Closing1.Button_detection.BUTTON_CAR.First_but_0 -> (junction 66860)
            (junction 66858) -> (junction 66861) [order 2]
            (junction 66859) -> (junction 66862) [order 2]
            (junction 66860) -> (junction 66863)
            (junction 66862) -> (junction 66861)
            (junction 66863) -> (junction 66862)
            (junction 66861) -> (junction 66866)
            Init_procedure.Closing_all_doors.Closing1.Button_detection.BUTTON_CAR.Button_CAR_1 -> (junction 66864)
            (junction 66864) -> Init_procedure.Closing_all_doors.Closing1.Button_detection.BUTTON_CAR.First_but_1 [order 1] : [FIRST_BUT && not(RPC1)]
            Init_procedure.Closing_all_doors.Closing1.Button_detection.BUTTON_CAR.First_but_1 -> (junction 66865)
            (junction 66864) -> (junction 66868) [order 2]
            (junction 66865) -> (junction 66869)
            (junction 66866) -> Init_procedure.Closing_all_doors.Closing1.Button_detection.BUTTON_CAR.Button_CAR_1 [order 1] : [P1]
            (junction 66866) -> (junction 66867) [order 2]
            (junction 66868) -> (junction 66867)
            (junction 66869) -> (junction 66868)
            (junction 66867) -> (junction 66870)
            (junction 66870) -> Init_procedure.Closing_all_doors.Closing1.Button_detection.BUTTON_CAR.Button_CAR_2 [order 1] : [P2]
            Init_procedure.Closing_all_doors.Closing1.Button_detection.BUTTON_CAR.Button_CAR_2 -> (junction 66871)
            (junction 66871) -> Init_procedure.Closing_all_doors.Closing1.Button_detection.BUTTON_CAR.First_but_2 [order 1] : [FIRST_BUT && not(RPC2)]
            Init_procedure.Closing_all_doors.Closing1.Button_detection.BUTTON_CAR.First_but_2 -> (junction 66872)
            (junction 66870) -> (junction 66873) [order 2]
            (junction 66871) -> (junction 66874) [order 2]
            (junction 66872) -> (junction 66875)
            (junction 66874) -> (junction 66873)
            (junction 66875) -> (junction 66874)
            (junction 66873) -> (junction 66876)
            (junction 66876) -> Init_procedure.Closing_all_doors.Closing1.Button_detection.BUTTON_CAR.Button_CAR_3 [order 1] : [P3]
            Init_procedure.Closing_all_doors.Closing1.Button_detection.BUTTON_CAR.Button_CAR_3 -> (junction 66877)
            (junction 66877) -> Init_procedure.Closing_all_doors.Closing1.Button_detection.BUTTON_CAR.First_but_3 [order 1] : [FIRST_BUT && not(RPC3)]
            Init_procedure.Closing_all_doors.Closing1.Button_detection.BUTTON_CAR.First_but_3 -> (junction 66878)
            (junction 66876) -> (junction 66879) [order 2]
            (junction 66877) -> (junction 66880) [order 2]
            (junction 66878) -> (junction 66881)
            (junction 66880) -> (junction 66879)
            (junction 66881) -> (junction 66880)
          state BUTTON_UP
            state Button_UP_0
              en:
              BUTTON_UP(1)=true;
              BUT_TEMP=0;
              LPS0=true;
              PUSHED=true;
              UPDATE=false;
              IN_LL=false; ET_LL=0;
            state First_but_0
              en:
              BUT_1=BUT_TEMP;
              FIRST_BUT=false;
            state Button_UP_1
              en:
              BUTTON_UP(2)=true;
              BUT_TEMP=1;
              LPS1=true;
              PUSHED=true;
              UPDATE=false;
              IN_LL=false; ET_LL=0;
            state First_but_1
              en:
              BUT_1=BUT_TEMP;
              FIRST_BUT=false;
            state Button_UP_2
              en:
              BUTTON_UP(3)=true;
              BUT_TEMP=2;
              LPS2=true;
              PUSHED=true;
              UPDATE=false;
              IN_LL=false; ET_LL=0;
            state First_but_2
              en:
              BUT_1=BUT_TEMP;
              FIRST_BUT=false;
            (junction 66931) -> Init_procedure.Closing_all_doors.Closing1.Button_detection.BUTTON_UP.Button_UP_0 [order 1] : [PS0]
            Init_procedure.Closing_all_doors.Closing1.Button_detection.BUTTON_UP.Button_UP_0 -> (junction 66932)
            (junction 66932) -> Init_procedure.Closing_all_doors.Closing1.Button_detection.BUTTON_UP.First_but_0 [order 1] : [FIRST_BUT && not(RPC0)]
            Init_procedure.Closing_all_doors.Closing1.Button_detection.BUTTON_UP.First_but_0 -> (junction 66933)
            (default) -> (junction 66931)
            (junction 66931) -> (junction 66936) [order 2]
            (junction 66932) -> (junction 66934) [order 2]
            (junction 66933) -> (junction 66935)
            (junction 66935) -> (junction 66934)
            (junction 66934) -> (junction 66936)
            (junction 66936) -> (junction 66937)
            (junction 66937) -> Init_procedure.Closing_all_doors.Closing1.Button_detection.BUTTON_UP.Button_UP_1 [order 1] : [PS1]
            Init_procedure.Closing_all_doors.Closing1.Button_detection.BUTTON_UP.Button_UP_1 -> (junction 66938)
            (junction 66938) -> Init_procedure.Closing_all_doors.Closing1.Button_detection.BUTTON_UP.First_but_1 [order 1] : [FIRST_BUT && not(RPC1)]
            Init_procedure.Closing_all_doors.Closing1.Button_detection.BUTTON_UP.First_but_1 -> (junction 66939)
            (junction 66937) -> (junction 66940) [order 2]
            (junction 66938) -> (junction 66941) [order 2]
            (junction 66939) -> (junction 66942)
            (junction 66941) -> (junction 66940)
            (junction 66942) -> (junction 66941)
            (junction 66940) -> (junction 66944)
            Init_procedure.Closing_all_doors.Closing1.Button_detection.BUTTON_UP.First_but_2 -> (junction 66943)
            (junction 66943) -> (junction 66948)
            (junction 66944) -> Init_procedure.Closing_all_doors.Closing1.Button_detection.BUTTON_UP.Button_UP_2 [order 1] : [PS2]
            Init_procedure.Closing_all_doors.Closing1.Button_detection.BUTTON_UP.Button_UP_2 -> (junction 66945)
            (junction 66945) -> Init_procedure.Closing_all_doors.Closing1.Button_detection.BUTTON_UP.First_but_2 [order 1] : [FIRST_BUT && not(RPC2)]
            (junction 66944) -> (junction 66946) [order 2]
            (junction 66945) -> (junction 66947) [order 2]
            (junction 66947) -> (junction 66946)
            (junction 66948) -> (junction 66947)
          state Max_Min_assignment
            state Min_but
              en:
              BUTTON=MIN_BUT;
            state Max_but
              en:
              BUTTON=MAX_BUT;
            state First_but
              en:
              BUTTON=BUT_1;
            state Max_but1
              en:
              MAX_BUT=2;
            state Max_but2
              en:
              MAX_BUT=1;
            state Max_but3
              en:
              MAX_BUT=0;
            state Min_but1
              en:
              MIN_BUT=1;
            state Min_but2
              en:
              MIN_BUT=2;
            state Min_but3
              en:
              MIN_BUT=3;
            state MAX
              en:
              MAX_BUT=BUT_TEMP;
            state MIN
              en:
              MIN_BUT=BUT_TEMP;
            state Updating_button_0
              en:
              BUTTON=MAX_BUT;
            state Updating_button_1
              en:
              BUTTON=MIN_BUT;
            (junction 66986) -> Init_procedure.Closing_all_doors.Closing1.Button_detection.Max_Min_assignment.Min_but [order 1] : [(MAX_BUT-FLOOR)>(FLOOR-MIN_BUT)]
            Init_procedure.Closing_all_doors.Closing1.Button_detection.Max_Min_assignment.Min_but -> (junction 66987)
            (junction 66988) -> (junction 66986) [order 1] : [not(FLAG_STOP) && MOTION==2 && FLAG==3]
            (default) -> (junction 66988)
            (junction 66986) -> (junction 66989) [order 2]
            (junction 66987) -> (junction 66990)
            (junction 66988) -> (junction 66991) [order 2]
            (junction 66989) -> Init_procedure.Closing_all_doors.Closing1.Button_detection.Max_Min_assignment.Max_but [order 1] : [(MAX_BUT-FLOOR)<(FLOOR-MIN_BUT)]
            Init_procedure.Closing_all_doors.Closing1.Button_detection.Max_Min_assignment.Max_but -> (junction 66990)
            (junction 66989) -> Init_procedure.Closing_all_doors.Closing1.Button_detection.Max_Min_assignment.First_but [order 2]
            (junction 66990) -> (junction 66993)
            Init_procedure.Closing_all_doors.Closing1.Button_detection.Max_Min_assignment.First_but -> (junction 66992)
            (junction 66992) -> (junction 66991)
            (junction 66993) -> (junction 66992)
            (junction 66991) -> (junction 66994)
            (junction 66995) -> (junction 66996) [order 1] : [MOTION==0]
                | {MOTION=1;
                | UPDATE=true;}
            (junction 66996) -> Init_procedure.Closing_all_doors.Closing1.Button_detection.Max_Min_assignment.Max_but1 [order 1] : [BUTTON_UP(2)]
            Init_procedure.Closing_all_doors.Closing1.Button_detection.Max_Min_assignment.Max_but1 -> (junction 66997)
            (junction 66994) -> (junction 66995) [order 1] : [BUTTON==FLOOR && EXTEND]
                | {EXTEND=false;}
            (junction 66994) -> (junction 67008) [order 2]
            (junction 66995) -> (junction 67000) [order 2]
            (junction 66996) -> (junction 66998) [order 2]
            (junction 66997) -> (junction 66999)
            (junction 66998) -> Init_procedure.Closing_all_doors.Closing1.Button_detection.Max_Min_assignment.Max_but2 [order 1] : [BUTTON_UP(1)]
            Init_procedure.Closing_all_doors.Closing1.Button_detection.Max_Min_assignment.Max_but2 -> (junction 66999)
            (junction 66998) -> Init_procedure.Closing_all_doors.Closing1.Button_detection.Max_Min_assignment.Max_but3 [order 2]
            (junction 66999) -> (junction 67002)
            Init_procedure.Closing_all_doors.Closing1.Button_detection.Max_Min_assignment.Max_but3 -> (junction 67001)
            (junction 67001) -> (junction 67000)
            (junction 67002) -> (junction 67001)
            (junction 67000) -> (junction 67003)
            (junction 67003) -> (junction 67004) [order 1] : [MOTION==1]
                | {MOTION=0;
                | UPDATE=true;}
            (junction 67004) -> Init_procedure.Closing_all_doors.Closing1.Button_detection.Max_Min_assignment.Min_but1 [order 1] : [BUTTON_DOWN(1)]
            Init_procedure.Closing_all_doors.Closing1.Button_detection.Max_Min_assignment.Min_but1 -> (junction 67005)
            (junction 67003) -> (junction 67009) [order 2]
            (junction 67004) -> (junction 67006) [order 2]
            (junction 67005) -> (junction 67007)
            (junction 67006) -> Init_procedure.Closing_all_doors.Closing1.Button_detection.Max_Min_assignment.Min_but2 [order 1] : [BUTTON_DOWN(2)]
            Init_procedure.Closing_all_doors.Closing1.Button_detection.Max_Min_assignment.Min_but2 -> (junction 67007)
            (junction 67006) -> Init_procedure.Closing_all_doors.Closing1.Button_detection.Max_Min_assignment.Min_but3 [order 2]
            (junction 67007) -> (junction 67011)
            Init_procedure.Closing_all_doors.Closing1.Button_detection.Max_Min_assignment.Min_but3 -> (junction 67010)
            (junction 67009) -> (junction 67008)
            (junction 67010) -> (junction 67009)
            (junction 67011) -> (junction 67010)
            (junction 67008) -> (junction 67013)
            Init_procedure.Closing_all_doors.Closing1.Button_detection.Max_Min_assignment.MAX -> (junction 67012)
            (junction 67013) -> (junction 67014) [order 1] : [PUSHED]
            (junction 67014) -> (junction 67015) [order 1] : [not(BUT_TEMP==FLOOR) || not(MOTION==2)]
            (junction 67015) -> Init_procedure.Closing_all_doors.Closing1.Button_detection.Max_Min_assignment.MAX [order 1] : [MAX_BUT<BUT_TEMP && not(UPDATE)]
            (junction 67012) -> (junction 67017)
            (junction 67013) -> (junction 67027) [order 2]
            (junction 67014) -> (junction 67020) [order 2]
            (junction 67015) -> (junction 67016) [order 2]
            (junction 67017) -> (junction 67016)
            (junction 67016) -> (junction 67018)
            (junction 67018) -> Init_procedure.Closing_all_doors.Closing1.Button_detection.Max_Min_assignment.MIN [order 1] : [MIN_BUT>BUT_TEMP && not(UPDATE)]
            Init_procedure.Closing_all_doors.Closing1.Button_detection.Max_Min_assignment.MIN -> (junction 67019)
            (junction 67018) -> (junction 67021) [order 2]
            (junction 67019) -> (junction 67022)
            (junction 67021) -> (junction 67020)
            (junction 67022) -> (junction 67021)
            (junction 67020) -> (junction 67023)
            (junction 67023) -> Init_procedure.Closing_all_doors.Closing1.Button_detection.Max_Min_assignment.Updating_button_0 [order 1] : [MOTION==0]
            Init_procedure.Closing_all_doors.Closing1.Button_detection.Max_Min_assignment.Updating_button_0 -> (junction 67024)
            (junction 67023) -> (junction 67025) [order 2]
            (junction 67024) -> (junction 67026)
            (junction 67025) -> Init_procedure.Closing_all_doors.Closing1.Button_detection.Max_Min_assignment.Updating_button_1 [order 1] : [MOTION==1]
            Init_procedure.Closing_all_doors.Closing1.Button_detection.Max_Min_assignment.Updating_button_1 -> (junction 67026)
            (junction 67025) -> (junction 67028) [order 2]
            (junction 67026) -> (junction 67029)
            (junction 67028) -> (junction 67027)
            (junction 67029) -> (junction 67028)
          state GoTo_PositionControl
            en:
            BUTTON=BUT_TEMP;
            FLAG=2;
          state Emergency
            en:
            FLAG_EMG=true;
            FLAG=4;
          state Timer_EME
            state Set_tmr
              en:
              Q_EME=true;
            state Counting
              en:
              ET_EME= ET_EME + 1;
              Q_EME=false;
            state Set
              en:
              IN_EME=true;
              PT_EME=3;
            (junction 67119) -> Init_procedure.Closing_all_doors.Closing1.Button_detection.Timer_EME.Set_tmr [order 1] : [ET_EME==PT_EME]
            Init_procedure.Closing_all_doors.Closing1.Button_detection.Timer_EME.Set_tmr -> (junction 67120)
            Init_procedure.Closing_all_doors.Closing1.Button_detection.Timer_EME.Counting -> (junction 67119)
            (junction 67119) -> (junction 67120) [order 2]
            (default) -> Init_procedure.Closing_all_doors.Closing1.Button_detection.Timer_EME.Set
            Init_procedure.Closing_all_doors.Closing1.Button_detection.Timer_EME.Set -> (junction 67121)
            (junction 67121) -> Init_procedure.Closing_all_doors.Closing1.Button_detection.Timer_EME.Counting [order 1] : [ET_EME<PT_EME]
            (junction 67121) -> (junction 67120) [order 2]
          state Not_Emergency
            en:
            IN_EME=false;
            ET_EME=0;
          state SwitchingOFF_LEDs
            en:
            LPD3=false;
            LPD2=false;
            LPS2=false;
            LPD1=false;
            LPS1=false;
            LPS0=false;
          (default) -> (junction 66720)
          (junction 66720) -> (junction 66721) [order 1] : [FLAG==1 && not(PUSHED)]
              | {BUTTON=FLOOR;
              | BUT_TEMP=BUTTON;
              | BUT_1=FLOOR;}
          (junction 66721) -> Init_procedure.Closing_all_doors.Closing1.Button_detection.Timer_LL [order 1] : [not(FLAG_STOP)]
          Init_procedure.Closing_all_doors.Closing1.Button_detection.Save_energy -> (junction 66722)
          Init_procedure.Closing_all_doors.Closing1.Button_detection.Timer_LL -> Init_procedure.Closing_all_doors.Closing1.Button_detection.Save_energy
          (junction 66721) -> (junction 66724) [order 2]
          (junction 66720) -> (junction 66723) [order 2]
          (junction 66722) -> (junction 66725)
          (junction 66724) -> (junction 66723)
          (junction 66725) -> (junction 66724)
          (junction 66723) -> Init_procedure.Closing_all_doors.Closing1.Button_detection.BUTTON_CAR
          Init_procedure.Closing_all_doors.Closing1.Button_detection.BUTTON_UP -> Init_procedure.Closing_all_doors.Closing1.Button_detection.BUTTON_DOWN
          Init_procedure.Closing_all_doors.Closing1.Button_detection.BUTTON_DOWN -> Init_procedure.Closing_all_doors.Closing1.Button_detection.Max_Min_assignment
          Init_procedure.Closing_all_doors.Closing1.Button_detection.Max_Min_assignment -> (junction 66726)
          Init_procedure.Closing_all_doors.Closing1.Button_detection.BUTTON_CAR -> Init_procedure.Closing_all_doors.Closing1.Button_detection.BUTTON_UP
          (junction 66726) -> (junction 66728)
          (junction 66728) -> (junction 66727)
          (junction 66727) -> (junction 66730)
          Init_procedure.Closing_all_doors.Closing1.Button_detection.GoTo_PositionControl -> (junction 66729)
          (junction 66730) -> (junction 66731) [order 1] : [FLAG==1]
          (junction 66731) -> Init_procedure.Closing_all_doors.Closing1.Button_detection.GoTo_PositionControl [order 1] : [PUSHED]
          (junction 66729) -> (junction 66733)
          (junction 66730) -> (junction 66741) [order 2]
          (junction 66731) -> (junction 66732) [order 2]
          (junction 66733) -> (junction 66732)
          (junction 66732) -> (junction 66735)
          Init_procedure.Closing_all_doors.Closing1.Button_detection.Emergency -> (junction 66734)
          (junction 66735) -> Init_procedure.Closing_all_doors.Closing1.Button_detection.Timer_EME [order 1] : [STOP]
              | {IN_LL=false; ET_LL=0;FLAG=1;}
          Init_procedure.Closing_all_doors.Closing1.Button_detection.Timer_EME -> (junction 66736)
          (junction 66736) -> Init_procedure.Closing_all_doors.Closing1.Button_detection.Emergency [order 1] : [Q_EME]
          (junction 66734) -> (junction 66738)
          (junction 66735) -> Init_procedure.Closing_all_doors.Closing1.Button_detection.Not_Emergency [order 2]
          (junction 66736) -> (junction 66737) [order 2]
          (junction 66738) -> (junction 66737)
          (junction 66737) -> (junction 66740)
          Init_procedure.Closing_all_doors.Closing1.Button_detection.Not_Emergency -> (junction 66740)
          Init_procedure.Closing_all_doors.Closing1.Button_detection.SwitchingOFF_LEDs -> (junction 66739)
          (junction 66740) -> Init_procedure.Closing_all_doors.Closing1.Button_detection.SwitchingOFF_LEDs [order 1] : [FLAG_STOP && FLAG==2]
          (junction 66739) -> (junction 66743)
          (junction 66740) -> (junction 66742) [order 2]
          (junction 66742) -> (junction 66741)
          (junction 66743) -> (junction 66742)
        state Extending
          en:
          EXTEND=true;
        state Stop_Closing
          en:
          CP1=false;
          FLAG_OD=false;
          OBS=false;
          ET_cl=0;
          IN_cl=false;
        state GoTo_PositionControl
          en: FLAG=2;
        state GoTo_BUttonDetection
          en:
          MOTION=2;
          MAX_BUT=0;
          MIN_BUT=3;
          PUSHED=false;
          FIRST_BUT=true;
          FLAG=1;
          UPDATE=false;
        state Closing1
          en:CP1=true;
        state Stop_Closing1
          en:CP1=false;
        Init_procedure.Closing_all_doors.Closing1.Reset -> Init_procedure.Closing_all_doors.Closing1.Timer_close
        (default) -> (junction 65282)
        (junction 65282) -> Init_procedure.Closing_all_doors.Closing1.Reset [order 1] : [not(FLAG==0) && not(FLAG==4)]
        Init_procedure.Closing_all_doors.Closing1.Timer_close -> (junction 65283)
        (junction 65283) -> Init_procedure.Closing_all_doors.Closing1.Closing [order 1] : [not(PC1)]
        Init_procedure.Closing_all_doors.Closing1.Button_detection -> (junction 65284)
        Init_procedure.Closing_all_doors.Closing1.Closing -> Init_procedure.Closing_all_doors.Closing1.Button_detection
        (junction 65282) -> (junction 65292) [order 2]
        (junction 65283) -> (junction 65285) [order 2]
        (junction 65284) -> (junction 65290)
        (junction 65285) -> Init_procedure.Closing_all_doors.Closing1.Extending [order 1] : [BUTTON==FLOOR]
        (junction 65285) -> (junction 65287) [order 2]
        Init_procedure.Closing_all_doors.Closing1.Extending -> (junction 65286)
        (junction 65286) -> (junction 65287)
        (junction 65287) -> Init_procedure.Closing_all_doors.Closing1.Stop_Closing
        Init_procedure.Closing_all_doors.Closing1.Stop_Closing -> (junction 65288)
        (junction 65288) -> Init_procedure.Closing_all_doors.Closing1.GoTo_PositionControl [order 2]
        (junction 65288) -> Init_procedure.Closing_all_doors.Closing1.GoTo_BUttonDetection [order 1] : [not(BUTTON_CAR(1) || BUTTON_CAR(2) || BUTTON_CAR(3) || BUTTON_CAR(4) || BUTTON_UP(1) || BUTTON_UP(2) || BUTTON_UP(3) || BUTTON_DOWN(2) || BUTTON_DOWN(3) || BUTTON_DOWN(4))]
        Init_procedure.Closing_all_doors.Closing1.GoTo_PositionControl -> (junction 65289)
        Init_procedure.Closing_all_doors.Closing1.GoTo_BUttonDetection -> (junction 65289)
        (junction 65289) -> (junction 65290)
        (junction 65290) -> (junction 65291)
        (junction 65291) -> (junction 65293)
        (junction 65292) -> Init_procedure.Closing_all_doors.Closing1.Closing1 [order 1] : [not(PC1)]
        Init_procedure.Closing_all_doors.Closing1.Closing1 -> (junction 65293)
        (junction 65292) -> Init_procedure.Closing_all_doors.Closing1.Stop_Closing1 [order 2]
        Init_procedure.Closing_all_doors.Closing1.Stop_Closing1 -> (junction 65293)
      state Closing2
        state Reset
          state Reset_0
            en:
            LPS0=false;
            BUTTON_CAR(1)=false;
            BUTTON_UP(1)=false;
          state Reset_1
            en:
            LPS1=false;
            LPD1=false;
            BUTTON_CAR(2)=false;
            BUTTON_UP(2)=false;
            BUTTON_DOWN(2)=false;
          state Reset_2
            en:
            LPS2=false;
            LPD2=false;
            BUTTON_CAR(3)=false;
            BUTTON_UP(3)=false;
            BUTTON_DOWN(3)=false;
          state Reset_3
            en:
            LPD3=false;
            BUTTON_CAR(4)=false;
            BUTTON_DOWN(4)=false;
          (default) -> (junction 65833)
          (junction 65833) -> Init_procedure.Closing_all_doors.Closing2.Reset.Reset_0 [order 1] : [FLOOR==0]
          Init_procedure.Closing_all_doors.Closing2.Reset.Reset_0 -> (junction 65834)
          (junction 65833) -> (junction 65835) [order 2]
          (junction 65834) -> (junction 65836)
          (junction 65835) -> Init_procedure.Closing_all_doors.Closing2.Reset.Reset_1 [order 1] : [FLOOR==1]
          Init_procedure.Closing_all_doors.Closing2.Reset.Reset_1 -> (junction 65836)
          (junction 65835) -> (junction 65837) [order 2]
          (junction 65836) -> (junction 65838)
          (junction 65837) -> Init_procedure.Closing_all_doors.Closing2.Reset.Reset_2 [order 1] : [FLOOR==2]
          Init_procedure.Closing_all_doors.Closing2.Reset.Reset_2 -> (junction 65838)
          (junction 65837) -> (junction 65839) [order 2]
          (junction 65838) -> (junction 65840)
          (junction 65839) -> Init_procedure.Closing_all_doors.Closing2.Reset.Reset_3 [order 1] : [FLOOR==3]
          Init_procedure.Closing_all_doors.Closing2.Reset.Reset_3 -> (junction 65840)
          (junction 65839) -> (junction 65841) [order 2]
          (junction 65840) -> (junction 65842)
          (junction 65842) -> (junction 65841)
        state Timer_close
          state Set_tmr
            en: Q_cl=true;
          state Set
            en:PT_cl=5;
            IN_cl=true;
          state Counting
            en:ET_cl = ET_cl + 1;
            Q_cl=false;
          (junction 65866) -> Init_procedure.Closing_all_doors.Closing2.Timer_close.Set_tmr [order 1] : [ET_cl==PT_cl]
          Init_procedure.Closing_all_doors.Closing2.Timer_close.Set_tmr -> (junction 65867)
          (default) -> Init_procedure.Closing_all_doors.Closing2.Timer_close.Set
          Init_procedure.Closing_all_doors.Closing2.Timer_close.Counting -> (junction 65866)
          (junction 65866) -> (junction 65867) [order 2]
          Init_procedure.Closing_all_doors.Closing2.Timer_close.Set -> (junction 65868)
          (junction 65868) -> Init_procedure.Closing_all_doors.Closing2.Timer_close.Counting [order 1] : [ET_cl<PT_cl]
          (junction 65868) -> (junction 65867) [order 2]
        state Closing
          en: CP2=Q_cl;
        state Button_detection
          state Save_energy
            en:
            LL=not(Q_LL);
          state Timer_LL
            state Set_tmr
              en:
              Q_LL=true;
            state Counting
              en:
              ET_LL= ET_LL + 1;
              Q_LL=false;
            state Set
              en:
              IN_LL=true;
              PT_LL=10;
            (junction 67204) -> Init_procedure.Closing_all_doors.Closing2.Button_detection.Timer_LL.Set_tmr [order 1] : [ET_LL==PT_LL]
            Init_procedure.Closing_all_doors.Closing2.Button_detection.Timer_LL.Set_tmr -> (junction 67205)
            Init_procedure.Closing_all_doors.Closing2.Button_detection.Timer_LL.Counting -> (junction 67204)
            (junction 67204) -> (junction 67205) [order 2]
            (default) -> Init_procedure.Closing_all_doors.Closing2.Button_detection.Timer_LL.Set
            Init_procedure.Closing_all_doors.Closing2.Button_detection.Timer_LL.Set -> (junction 67206)
            (junction 67206) -> Init_procedure.Closing_all_doors.Closing2.Button_detection.Timer_LL.Counting [order 1] : [ET_LL<PT_LL]
            (junction 67206) -> (junction 67205) [order 2]
          state BUTTON_DOWN
            state Button_DOWN_1
              en:
              BUTTON_DOWN(2)=true;
              BUT_TEMP=1;
              LPD1=true;
              PUSHED=true;
              UPDATE=false;
              IN_LL=false; ET_LL=0;
            state First_but_1
              en:
              BUT_1=BUT_TEMP;
              FIRST_BUT=false;
            state Button_DOWN_2
              en:
              BUTTON_DOWN(3)=true;
              BUT_TEMP=2;
              LPD2=true;
              PUSHED=true;
              UPDATE=false;
              IN_LL=false; ET_LL=0;
            state First_but_2
              en:
              BUT_1=BUT_TEMP;
              FIRST_BUT=false;
            state Button_DOWN_3
              en:
              BUTTON_DOWN(4)=true;
              BUT_TEMP=3;
              LPD3=true;
              PUSHED=true;
              UPDATE=false;
              IN_LL=false; ET_LL=0;
            state First_but_3
              en:
              BUT_1=BUT_TEMP;
              FIRST_BUT=false;
            (default) -> (junction 67219)
            (junction 67219) -> Init_procedure.Closing_all_doors.Closing2.Button_detection.BUTTON_DOWN.Button_DOWN_1 [order 1] : [PD1]
            Init_procedure.Closing_all_doors.Closing2.Button_detection.BUTTON_DOWN.Button_DOWN_1 -> (junction 67220)
            (junction 67220) -> Init_procedure.Closing_all_doors.Closing2.Button_detection.BUTTON_DOWN.First_but_1 [order 1] : [FIRST_BUT && not(RPC1)]
            Init_procedure.Closing_all_doors.Closing2.Button_detection.BUTTON_DOWN.First_but_1 -> (junction 67221)
            (junction 67219) -> (junction 67222) [order 2]
            (junction 67220) -> (junction 67223) [order 2]
            (junction 67221) -> (junction 67224)
            (junction 67223) -> (junction 67222)
            (junction 67224) -> (junction 67223)
            (junction 67222) -> (junction 67225)
            (junction 67225) -> Init_procedure.Closing_all_doors.Closing2.Button_detection.BUTTON_DOWN.Button_DOWN_2 [order 1] : [PD2]
            Init_procedure.Closing_all_doors.Closing2.Button_detection.BUTTON_DOWN.Button_DOWN_2 -> (junction 67226)
            (junction 67226) -> Init_procedure.Closing_all_doors.Closing2.Button_detection.BUTTON_DOWN.First_but_2 [order 1] : [FIRST_BUT && not(RPC2)]
            Init_procedure.Closing_all_doors.Closing2.Button_detection.BUTTON_DOWN.First_but_2 -> (junction 67227)
            (junction 67225) -> (junction 67228) [order 2]
            (junction 67226) -> (junction 67229) [order 2]
            (junction 67227) -> (junction 67230)
            (junction 67229) -> (junction 67228)
            (junction 67230) -> (junction 67229)
            (junction 67228) -> (junction 67231)
            (junction 67231) -> Init_procedure.Closing_all_doors.Closing2.Button_detection.BUTTON_DOWN.Button_DOWN_3 [order 1] : [PD3]
            Init_procedure.Closing_all_doors.Closing2.Button_detection.BUTTON_DOWN.Button_DOWN_3 -> (junction 67232)
            (junction 67232) -> Init_procedure.Closing_all_doors.Closing2.Button_detection.BUTTON_DOWN.First_but_3 [order 1] : [FIRST_BUT && not(RPC3)]
            Init_procedure.Closing_all_doors.Closing2.Button_detection.BUTTON_DOWN.First_but_3 -> (junction 67233)
            (junction 67231) -> (junction 67234) [order 2]
            (junction 67232) -> (junction 67235) [order 2]
            (junction 67233) -> (junction 67236)
            (junction 67235) -> (junction 67234)
            (junction 67236) -> (junction 67235)
          state BUTTON_CAR
            state Button_CAR_0
              en:
              BUTTON_CAR(1)=true;
              BUT_TEMP=0;
              LPC0=true;
              PUSHED=true;
              UPDATE=false;
              IN_LL=false; ET_LL=0;
            state First_but_0
              en:
              BUT_1=BUT_TEMP;
              FIRST_BUT=false;
            state Button_CAR_1
              en:
              BUTTON_CAR(2)=true;
              BUT_TEMP=1;
              LPC1=true;
              PUSHED=true;
              UPDATE=false;
              IN_LL=false; ET_LL=0;
            state First_but_1
              en:
              BUT_1=BUT_TEMP;
              FIRST_BUT=false;
            state Button_CAR_2
              en:
              BUTTON_CAR(3)=true;
              BUT_TEMP=2;
              LPC2=true;
              PUSHED=true;
              UPDATE=false;
              IN_LL=false; ET_LL=0;
            state First_but_2
              en:
              BUT_1=BUT_TEMP;
              FIRST_BUT=false;
            state Button_CAR_3
              en:
              BUTTON_CAR(4)=true;
              BUT_TEMP=3;
              LPC3=true;
              PUSHED=true;
              UPDATE=false;
              IN_LL=false; ET_LL=0;
            state First_but_3
              en:
              BUT_1=BUT_TEMP;
              FIRST_BUT=false;
            (default) -> (junction 67274)
            (junction 67274) -> Init_procedure.Closing_all_doors.Closing2.Button_detection.BUTTON_CAR.Button_CAR_0 [order 1] : [P0]
            Init_procedure.Closing_all_doors.Closing2.Button_detection.BUTTON_CAR.Button_CAR_0 -> (junction 67275)
            (junction 67275) -> Init_procedure.Closing_all_doors.Closing2.Button_detection.BUTTON_CAR.First_but_0 [order 1] : [FIRST_BUT && not(RPC0)]
            Init_procedure.Closing_all_doors.Closing2.Button_detection.BUTTON_CAR.First_but_0 -> (junction 67276)
            (junction 67274) -> (junction 67277) [order 2]
            (junction 67275) -> (junction 67278) [order 2]
            (junction 67276) -> (junction 67279)
            (junction 67278) -> (junction 67277)
            (junction 67279) -> (junction 67278)
            (junction 67277) -> (junction 67282)
            Init_procedure.Closing_all_doors.Closing2.Button_detection.BUTTON_CAR.Button_CAR_1 -> (junction 67280)
            (junction 67280) -> Init_procedure.Closing_all_doors.Closing2.Button_detection.BUTTON_CAR.First_but_1 [order 1] : [FIRST_BUT && not(RPC1)]
            Init_procedure.Closing_all_doors.Closing2.Button_detection.BUTTON_CAR.First_but_1 -> (junction 67281)
            (junction 67280) -> (junction 67284) [order 2]
            (junction 67281) -> (junction 67285)
            (junction 67282) -> Init_procedure.Closing_all_doors.Closing2.Button_detection.BUTTON_CAR.Button_CAR_1 [order 1] : [P1]
            (junction 67282) -> (junction 67283) [order 2]
            (junction 67284) -> (junction 67283)
            (junction 67285) -> (junction 67284)
            (junction 67283) -> (junction 67286)
            (junction 67286) -> Init_procedure.Closing_all_doors.Closing2.Button_detection.BUTTON_CAR.Button_CAR_2 [order 1] : [P2]
            Init_procedure.Closing_all_doors.Closing2.Button_detection.BUTTON_CAR.Button_CAR_2 -> (junction 67287)
            (junction 67287) -> Init_procedure.Closing_all_doors.Closing2.Button_detection.BUTTON_CAR.First_but_2 [order 1] : [FIRST_BUT && not(RPC2)]
            Init_procedure.Closing_all_doors.Closing2.Button_detection.BUTTON_CAR.First_but_2 -> (junction 67288)
            (junction 67286) -> (junction 67289) [order 2]
            (junction 67287) -> (junction 67290) [order 2]
            (junction 67288) -> (junction 67291)
            (junction 67290) -> (junction 67289)
            (junction 67291) -> (junction 67290)
            (junction 67289) -> (junction 67292)
            (junction 67292) -> Init_procedure.Closing_all_doors.Closing2.Button_detection.BUTTON_CAR.Button_CAR_3 [order 1] : [P3]
            Init_procedure.Closing_all_doors.Closing2.Button_detection.BUTTON_CAR.Button_CAR_3 -> (junction 67293)
            (junction 67293) -> Init_procedure.Closing_all_doors.Closing2.Button_detection.BUTTON_CAR.First_but_3 [order 1] : [FIRST_BUT && not(RPC3)]
            Init_procedure.Closing_all_doors.Closing2.Button_detection.BUTTON_CAR.First_but_3 -> (junction 67294)
            (junction 67292) -> (junction 67295) [order 2]
            (junction 67293) -> (junction 67296) [order 2]
            (junction 67294) -> (junction 67297)
            (junction 67296) -> (junction 67295)
            (junction 67297) -> (junction 67296)
          state BUTTON_UP
            state Button_UP_0
              en:
              BUTTON_UP(1)=true;
              BUT_TEMP=0;
              LPS0=true;
              PUSHED=true;
              UPDATE=false;
              IN_LL=false; ET_LL=0;
            state First_but_0
              en:
              BUT_1=BUT_TEMP;
              FIRST_BUT=false;
            state Button_UP_1
              en:
              BUTTON_UP(2)=true;
              BUT_TEMP=1;
              LPS1=true;
              PUSHED=true;
              UPDATE=false;
              IN_LL=false; ET_LL=0;
            state First_but_1
              en:
              BUT_1=BUT_TEMP;
              FIRST_BUT=false;
            state Button_UP_2
              en:
              BUTTON_UP(3)=true;
              BUT_TEMP=2;
              LPS2=true;
              PUSHED=true;
              UPDATE=false;
              IN_LL=false; ET_LL=0;
            state First_but_2
              en:
              BUT_1=BUT_TEMP;
              FIRST_BUT=false;
            (junction 67347) -> Init_procedure.Closing_all_doors.Closing2.Button_detection.BUTTON_UP.Button_UP_0 [order 1] : [PS0]
            Init_procedure.Closing_all_doors.Closing2.Button_detection.BUTTON_UP.Button_UP_0 -> (junction 67348)
            (junction 67348) -> Init_procedure.Closing_all_doors.Closing2.Button_detection.BUTTON_UP.First_but_0 [order 1] : [FIRST_BUT && not(RPC0)]
            Init_procedure.Closing_all_doors.Closing2.Button_detection.BUTTON_UP.First_but_0 -> (junction 67349)
            (default) -> (junction 67347)
            (junction 67347) -> (junction 67352) [order 2]
            (junction 67348) -> (junction 67350) [order 2]
            (junction 67349) -> (junction 67351)
            (junction 67351) -> (junction 67350)
            (junction 67350) -> (junction 67352)
            (junction 67352) -> (junction 67353)
            (junction 67353) -> Init_procedure.Closing_all_doors.Closing2.Button_detection.BUTTON_UP.Button_UP_1 [order 1] : [PS1]
            Init_procedure.Closing_all_doors.Closing2.Button_detection.BUTTON_UP.Button_UP_1 -> (junction 67354)
            (junction 67354) -> Init_procedure.Closing_all_doors.Closing2.Button_detection.BUTTON_UP.First_but_1 [order 1] : [FIRST_BUT && not(RPC1)]
            Init_procedure.Closing_all_doors.Closing2.Button_detection.BUTTON_UP.First_but_1 -> (junction 67355)
            (junction 67353) -> (junction 67356) [order 2]
            (junction 67354) -> (junction 67357) [order 2]
            (junction 67355) -> (junction 67358)
            (junction 67357) -> (junction 67356)
            (junction 67358) -> (junction 67357)
            (junction 67356) -> (junction 67360)
            Init_procedure.Closing_all_doors.Closing2.Button_detection.BUTTON_UP.First_but_2 -> (junction 67359)
            (junction 67359) -> (junction 67364)
            (junction 67360) -> Init_procedure.Closing_all_doors.Closing2.Button_detection.BUTTON_UP.Button_UP_2 [order 1] : [PS2]
            Init_procedure.Closing_all_doors.Closing2.Button_detection.BUTTON_UP.Button_UP_2 -> (junction 67361)
            (junction 67361) -> Init_procedure.Closing_all_doors.Closing2.Button_detection.BUTTON_UP.First_but_2 [order 1] : [FIRST_BUT && not(RPC2)]
            (junction 67360) -> (junction 67362) [order 2]
            (junction 67361) -> (junction 67363) [order 2]
            (junction 67363) -> (junction 67362)
            (junction 67364) -> (junction 67363)
          state Max_Min_assignment
            state Min_but
              en:
              BUTTON=MIN_BUT;
            state Max_but
              en:
              BUTTON=MAX_BUT;
            state First_but
              en:
              BUTTON=BUT_1;
            state Max_but1
              en:
              MAX_BUT=2;
            state Max_but2
              en:
              MAX_BUT=1;
            state Max_but3
              en:
              MAX_BUT=0;
            state Min_but1
              en:
              MIN_BUT=1;
            state Min_but2
              en:
              MIN_BUT=2;
            state Min_but3
              en:
              MIN_BUT=3;
            state MAX
              en:
              MAX_BUT=BUT_TEMP;
            state MIN
              en:
              MIN_BUT=BUT_TEMP;
            state Updating_button_0
              en:
              BUTTON=MAX_BUT;
            state Updating_button_1
              en:
              BUTTON=MIN_BUT;
            (junction 67402) -> Init_procedure.Closing_all_doors.Closing2.Button_detection.Max_Min_assignment.Min_but [order 1] : [(MAX_BUT-FLOOR)>(FLOOR-MIN_BUT)]
            Init_procedure.Closing_all_doors.Closing2.Button_detection.Max_Min_assignment.Min_but -> (junction 67403)
            (junction 67404) -> (junction 67402) [order 1] : [not(FLAG_STOP) && MOTION==2 && FLAG==3]
            (default) -> (junction 67404)
            (junction 67402) -> (junction 67405) [order 2]
            (junction 67403) -> (junction 67406)
            (junction 67404) -> (junction 67407) [order 2]
            (junction 67405) -> Init_procedure.Closing_all_doors.Closing2.Button_detection.Max_Min_assignment.Max_but [order 1] : [(MAX_BUT-FLOOR)<(FLOOR-MIN_BUT)]
            Init_procedure.Closing_all_doors.Closing2.Button_detection.Max_Min_assignment.Max_but -> (junction 67406)
            (junction 67405) -> Init_procedure.Closing_all_doors.Closing2.Button_detection.Max_Min_assignment.First_but [order 2]
            (junction 67406) -> (junction 67409)
            Init_procedure.Closing_all_doors.Closing2.Button_detection.Max_Min_assignment.First_but -> (junction 67408)
            (junction 67408) -> (junction 67407)
            (junction 67409) -> (junction 67408)
            (junction 67407) -> (junction 67410)
            (junction 67411) -> (junction 67412) [order 1] : [MOTION==0]
                | {MOTION=1;
                | UPDATE=true;}
            (junction 67412) -> Init_procedure.Closing_all_doors.Closing2.Button_detection.Max_Min_assignment.Max_but1 [order 1] : [BUTTON_UP(2)]
            Init_procedure.Closing_all_doors.Closing2.Button_detection.Max_Min_assignment.Max_but1 -> (junction 67413)
            (junction 67410) -> (junction 67411) [order 1] : [BUTTON==FLOOR && EXTEND]
                | {EXTEND=false;}
            (junction 67410) -> (junction 67424) [order 2]
            (junction 67411) -> (junction 67416) [order 2]
            (junction 67412) -> (junction 67414) [order 2]
            (junction 67413) -> (junction 67415)
            (junction 67414) -> Init_procedure.Closing_all_doors.Closing2.Button_detection.Max_Min_assignment.Max_but2 [order 1] : [BUTTON_UP(1)]
            Init_procedure.Closing_all_doors.Closing2.Button_detection.Max_Min_assignment.Max_but2 -> (junction 67415)
            (junction 67414) -> Init_procedure.Closing_all_doors.Closing2.Button_detection.Max_Min_assignment.Max_but3 [order 2]
            (junction 67415) -> (junction 67418)
            Init_procedure.Closing_all_doors.Closing2.Button_detection.Max_Min_assignment.Max_but3 -> (junction 67417)
            (junction 67417) -> (junction 67416)
            (junction 67418) -> (junction 67417)
            (junction 67416) -> (junction 67419)
            (junction 67419) -> (junction 67420) [order 1] : [MOTION==1]
                | {MOTION=0;
                | UPDATE=true;}
            (junction 67420) -> Init_procedure.Closing_all_doors.Closing2.Button_detection.Max_Min_assignment.Min_but1 [order 1] : [BUTTON_DOWN(1)]
            Init_procedure.Closing_all_doors.Closing2.Button_detection.Max_Min_assignment.Min_but1 -> (junction 67421)
            (junction 67419) -> (junction 67425) [order 2]
            (junction 67420) -> (junction 67422) [order 2]
            (junction 67421) -> (junction 67423)
            (junction 67422) -> Init_procedure.Closing_all_doors.Closing2.Button_detection.Max_Min_assignment.Min_but2 [order 1] : [BUTTON_DOWN(2)]
            Init_procedure.Closing_all_doors.Closing2.Button_detection.Max_Min_assignment.Min_but2 -> (junction 67423)
            (junction 67422) -> Init_procedure.Closing_all_doors.Closing2.Button_detection.Max_Min_assignment.Min_but3 [order 2]
            (junction 67423) -> (junction 67427)
            Init_procedure.Closing_all_doors.Closing2.Button_detection.Max_Min_assignment.Min_but3 -> (junction 67426)
            (junction 67425) -> (junction 67424)
            (junction 67426) -> (junction 67425)
            (junction 67427) -> (junction 67426)
            (junction 67424) -> (junction 67429)
            Init_procedure.Closing_all_doors.Closing2.Button_detection.Max_Min_assignment.MAX -> (junction 67428)
            (junction 67429) -> (junction 67430) [order 1] : [PUSHED]
            (junction 67430) -> (junction 67431) [order 1] : [not(BUT_TEMP==FLOOR) || not(MOTION==2)]
            (junction 67431) -> Init_procedure.Closing_all_doors.Closing2.Button_detection.Max_Min_assignment.MAX [order 1] : [MAX_BUT<BUT_TEMP && not(UPDATE)]
            (junction 67428) -> (junction 67433)
            (junction 67429) -> (junction 67443) [order 2]
            (junction 67430) -> (junction 67436) [order 2]
            (junction 67431) -> (junction 67432) [order 2]
            (junction 67433) -> (junction 67432)
            (junction 67432) -> (junction 67434)
            (junction 67434) -> Init_procedure.Closing_all_doors.Closing2.Button_detection.Max_Min_assignment.MIN [order 1] : [MIN_BUT>BUT_TEMP && not(UPDATE)]
            Init_procedure.Closing_all_doors.Closing2.Button_detection.Max_Min_assignment.MIN -> (junction 67435)
            (junction 67434) -> (junction 67437) [order 2]
            (junction 67435) -> (junction 67438)
            (junction 67437) -> (junction 67436)
            (junction 67438) -> (junction 67437)
            (junction 67436) -> (junction 67439)
            (junction 67439) -> Init_procedure.Closing_all_doors.Closing2.Button_detection.Max_Min_assignment.Updating_button_0 [order 1] : [MOTION==0]
            Init_procedure.Closing_all_doors.Closing2.Button_detection.Max_Min_assignment.Updating_button_0 -> (junction 67440)
            (junction 67439) -> (junction 67441) [order 2]
            (junction 67440) -> (junction 67442)
            (junction 67441) -> Init_procedure.Closing_all_doors.Closing2.Button_detection.Max_Min_assignment.Updating_button_1 [order 1] : [MOTION==1]
            Init_procedure.Closing_all_doors.Closing2.Button_detection.Max_Min_assignment.Updating_button_1 -> (junction 67442)
            (junction 67441) -> (junction 67444) [order 2]
            (junction 67442) -> (junction 67445)
            (junction 67444) -> (junction 67443)
            (junction 67445) -> (junction 67444)
          state GoTo_PositionControl
            en:
            BUTTON=BUT_TEMP;
            FLAG=2;
          state Emergency
            en:
            FLAG_EMG=true;
            FLAG=4;
          state Timer_EME
            state Set_tmr
              en:
              Q_EME=true;
            state Counting
              en:
              ET_EME= ET_EME + 1;
              Q_EME=false;
            state Set
              en:
              IN_EME=true;
              PT_EME=3;
            (junction 67535) -> Init_procedure.Closing_all_doors.Closing2.Button_detection.Timer_EME.Set_tmr [order 1] : [ET_EME==PT_EME]
            Init_procedure.Closing_all_doors.Closing2.Button_detection.Timer_EME.Set_tmr -> (junction 67536)
            Init_procedure.Closing_all_doors.Closing2.Button_detection.Timer_EME.Counting -> (junction 67535)
            (junction 67535) -> (junction 67536) [order 2]
            (default) -> Init_procedure.Closing_all_doors.Closing2.Button_detection.Timer_EME.Set
            Init_procedure.Closing_all_doors.Closing2.Button_detection.Timer_EME.Set -> (junction 67537)
            (junction 67537) -> Init_procedure.Closing_all_doors.Closing2.Button_detection.Timer_EME.Counting [order 1] : [ET_EME<PT_EME]
            (junction 67537) -> (junction 67536) [order 2]
          state Not_Emergency
            en:
            IN_EME=false;
            ET_EME=0;
          state SwitchingOFF_LEDs
            en:
            LPD3=false;
            LPD2=false;
            LPS2=false;
            LPD1=false;
            LPS1=false;
            LPS0=false;
          (default) -> (junction 67136)
          (junction 67136) -> (junction 67137) [order 1] : [FLAG==1 && not(PUSHED)]
              | {BUTTON=FLOOR;
              | BUT_TEMP=BUTTON;
              | BUT_1=FLOOR;}
          (junction 67137) -> Init_procedure.Closing_all_doors.Closing2.Button_detection.Timer_LL [order 1] : [not(FLAG_STOP)]
          Init_procedure.Closing_all_doors.Closing2.Button_detection.Save_energy -> (junction 67138)
          Init_procedure.Closing_all_doors.Closing2.Button_detection.Timer_LL -> Init_procedure.Closing_all_doors.Closing2.Button_detection.Save_energy
          (junction 67137) -> (junction 67140) [order 2]
          (junction 67136) -> (junction 67139) [order 2]
          (junction 67138) -> (junction 67141)
          (junction 67140) -> (junction 67139)
          (junction 67141) -> (junction 67140)
          (junction 67139) -> Init_procedure.Closing_all_doors.Closing2.Button_detection.BUTTON_CAR
          Init_procedure.Closing_all_doors.Closing2.Button_detection.BUTTON_UP -> Init_procedure.Closing_all_doors.Closing2.Button_detection.BUTTON_DOWN
          Init_procedure.Closing_all_doors.Closing2.Button_detection.BUTTON_DOWN -> Init_procedure.Closing_all_doors.Closing2.Button_detection.Max_Min_assignment
          Init_procedure.Closing_all_doors.Closing2.Button_detection.Max_Min_assignment -> (junction 67142)
          Init_procedure.Closing_all_doors.Closing2.Button_detection.BUTTON_CAR -> Init_procedure.Closing_all_doors.Closing2.Button_detection.BUTTON_UP
          (junction 67142) -> (junction 67144)
          (junction 67144) -> (junction 67143)
          (junction 67143) -> (junction 67146)
          Init_procedure.Closing_all_doors.Closing2.Button_detection.GoTo_PositionControl -> (junction 67145)
          (junction 67146) -> (junction 67147) [order 1] : [FLAG==1]
          (junction 67147) -> Init_procedure.Closing_all_doors.Closing2.Button_detection.GoTo_PositionControl [order 1] : [PUSHED]
          (junction 67145) -> (junction 67149)
          (junction 67146) -> (junction 67157) [order 2]
          (junction 67147) -> (junction 67148) [order 2]
          (junction 67149) -> (junction 67148)
          (junction 67148) -> (junction 67151)
          Init_procedure.Closing_all_doors.Closing2.Button_detection.Emergency -> (junction 67150)
          (junction 67151) -> Init_procedure.Closing_all_doors.Closing2.Button_detection.Timer_EME [order 1] : [STOP]
              | {IN_LL=false; ET_LL=0;FLAG=1;}
          Init_procedure.Closing_all_doors.Closing2.Button_detection.Timer_EME -> (junction 67152)
          (junction 67152) -> Init_procedure.Closing_all_doors.Closing2.Button_detection.Emergency [order 1] : [Q_EME]
          (junction 67150) -> (junction 67154)
          (junction 67151) -> Init_procedure.Closing_all_doors.Closing2.Button_detection.Not_Emergency [order 2]
          (junction 67152) -> (junction 67153) [order 2]
          (junction 67154) -> (junction 67153)
          (junction 67153) -> (junction 67156)
          Init_procedure.Closing_all_doors.Closing2.Button_detection.Not_Emergency -> (junction 67156)
          Init_procedure.Closing_all_doors.Closing2.Button_detection.SwitchingOFF_LEDs -> (junction 67155)
          (junction 67156) -> Init_procedure.Closing_all_doors.Closing2.Button_detection.SwitchingOFF_LEDs [order 1] : [FLAG_STOP && FLAG==2]
          (junction 67155) -> (junction 67159)
          (junction 67156) -> (junction 67158) [order 2]
          (junction 67158) -> (junction 67157)
          (junction 67159) -> (junction 67158)
        state Extending
          en:
          EXTEND=true;
        state Stop_Closing
          en:
          CP2=false;
          FLAG_OD=false;
          OBS=false;
          ET_cl=0;
          IN_cl=false;
        state GoTo_PositionControl
          en: FLAG=2;
        state GoTo_BUttonDetection
          en:
          MOTION=2;
          MAX_BUT=0;
          MIN_BUT=3;
          PUSHED=false;
          FIRST_BUT=true;
          FLAG=1;
          UPDATE=false;
        state Closing1
          en:CP2=true;
        state Stop_Closing1
          en:CP2=false;
        Init_procedure.Closing_all_doors.Closing2.Reset -> Init_procedure.Closing_all_doors.Closing2.Timer_close
        (default) -> (junction 65793)
        (junction 65793) -> Init_procedure.Closing_all_doors.Closing2.Reset [order 1] : [not(FLAG==0) && not(FLAG==4)]
        Init_procedure.Closing_all_doors.Closing2.Timer_close -> (junction 65794)
        (junction 65794) -> Init_procedure.Closing_all_doors.Closing2.Closing [order 1] : [not(PC2)]
        Init_procedure.Closing_all_doors.Closing2.Button_detection -> (junction 65795)
        Init_procedure.Closing_all_doors.Closing2.Closing -> Init_procedure.Closing_all_doors.Closing2.Button_detection
        (junction 65793) -> (junction 65803) [order 2]
        (junction 65794) -> (junction 65796) [order 2]
        (junction 65795) -> (junction 65801)
        (junction 65796) -> Init_procedure.Closing_all_doors.Closing2.Extending [order 1] : [BUTTON==FLOOR]
        (junction 65796) -> (junction 65798) [order 2]
        Init_procedure.Closing_all_doors.Closing2.Extending -> (junction 65797)
        (junction 65797) -> (junction 65798)
        (junction 65798) -> Init_procedure.Closing_all_doors.Closing2.Stop_Closing
        Init_procedure.Closing_all_doors.Closing2.Stop_Closing -> (junction 65799)
        (junction 65799) -> Init_procedure.Closing_all_doors.Closing2.GoTo_PositionControl [order 2]
        (junction 65799) -> Init_procedure.Closing_all_doors.Closing2.GoTo_BUttonDetection [order 1] : [not(BUTTON_CAR(1) || BUTTON_CAR(2) || BUTTON_CAR(3) || BUTTON_CAR(4) || BUTTON_UP(1) || BUTTON_UP(2) || BUTTON_UP(3) || BUTTON_DOWN(2) || BUTTON_DOWN(3) || BUTTON_DOWN(4))]
        Init_procedure.Closing_all_doors.Closing2.GoTo_PositionControl -> (junction 65800)
        Init_procedure.Closing_all_doors.Closing2.GoTo_BUttonDetection -> (junction 65800)
        (junction 65800) -> (junction 65801)
        (junction 65801) -> (junction 65802)
        (junction 65802) -> (junction 65804)
        (junction 65803) -> Init_procedure.Closing_all_doors.Closing2.Closing1 [order 1] : [not(PC2)]
        Init_procedure.Closing_all_doors.Closing2.Closing1 -> (junction 65804)
        (junction 65803) -> Init_procedure.Closing_all_doors.Closing2.Stop_Closing1 [order 2]
        Init_procedure.Closing_all_doors.Closing2.Stop_Closing1 -> (junction 65804)
      state Closing3
        state Reset
          state Reset_0
            en:
            LPS0=false;
            BUTTON_CAR(1)=false;
            BUTTON_UP(1)=false;
          state Reset_1
            en:
            LPS1=false;
            LPD1=false;
            BUTTON_CAR(2)=false;
            BUTTON_UP(2)=false;
            BUTTON_DOWN(2)=false;
          state Reset_2
            en:
            LPS2=false;
            LPD2=false;
            BUTTON_CAR(3)=false;
            BUTTON_UP(3)=false;
            BUTTON_DOWN(3)=false;
          state Reset_3
            en:
            LPD3=false;
            BUTTON_CAR(4)=false;
            BUTTON_DOWN(4)=false;
          (default) -> (junction 67592)
          (junction 67592) -> Init_procedure.Closing_all_doors.Closing3.Reset.Reset_0 [order 1] : [FLOOR==0]
          Init_procedure.Closing_all_doors.Closing3.Reset.Reset_0 -> (junction 67593)
          (junction 67592) -> (junction 67594) [order 2]
          (junction 67593) -> (junction 67595)
          (junction 67594) -> Init_procedure.Closing_all_doors.Closing3.Reset.Reset_1 [order 1] : [FLOOR==1]
          Init_procedure.Closing_all_doors.Closing3.Reset.Reset_1 -> (junction 67595)
          (junction 67594) -> (junction 67596) [order 2]
          (junction 67595) -> (junction 67597)
          (junction 67596) -> Init_procedure.Closing_all_doors.Closing3.Reset.Reset_2 [order 1] : [FLOOR==2]
          Init_procedure.Closing_all_doors.Closing3.Reset.Reset_2 -> (junction 67597)
          (junction 67596) -> (junction 67598) [order 2]
          (junction 67597) -> (junction 67599)
          (junction 67598) -> Init_procedure.Closing_all_doors.Closing3.Reset.Reset_3 [order 1] : [FLOOR==3]
          Init_procedure.Closing_all_doors.Closing3.Reset.Reset_3 -> (junction 67599)
          (junction 67598) -> (junction 67600) [order 2]
          (junction 67599) -> (junction 67601)
          (junction 67601) -> (junction 67600)
        state Timer_close
          state Set_tmr
            en: Q_cl=true;
          state Set
            en:PT_cl=5;
            IN_cl=true;
          state Counting
            en:ET_cl = ET_cl + 1;
            Q_cl=false;
          (junction 67625) -> Init_procedure.Closing_all_doors.Closing3.Timer_close.Set_tmr [order 1] : [ET_cl==PT_cl]
          Init_procedure.Closing_all_doors.Closing3.Timer_close.Set_tmr -> (junction 67626)
          (default) -> Init_procedure.Closing_all_doors.Closing3.Timer_close.Set
          Init_procedure.Closing_all_doors.Closing3.Timer_close.Counting -> (junction 67625)
          (junction 67625) -> (junction 67626) [order 2]
          Init_procedure.Closing_all_doors.Closing3.Timer_close.Set -> (junction 67627)
          (junction 67627) -> Init_procedure.Closing_all_doors.Closing3.Timer_close.Counting [order 1] : [ET_cl<PT_cl]
          (junction 67627) -> (junction 67626) [order 2]
        state Closing
          en: CP2=Q_cl;
        state Button_detection
          state Save_energy
            en:
            LL=not(Q_LL);
          state Timer_LL
            state Set_tmr
              en:
              Q_LL=true;
            state Counting
              en:
              ET_LL= ET_LL + 1;
              Q_LL=false;
            state Set
              en:
              IN_LL=true;
              PT_LL=10;
            (junction 67709) -> Init_procedure.Closing_all_doors.Closing3.Button_detection.Timer_LL.Set_tmr [order 1] : [ET_LL==PT_LL]
            Init_procedure.Closing_all_doors.Closing3.Button_detection.Timer_LL.Set_tmr -> (junction 67710)
            Init_procedure.Closing_all_doors.Closing3.Button_detection.Timer_LL.Counting -> (junction 67709)
            (junction 67709) -> (junction 67710) [order 2]
            (default) -> Init_procedure.Closing_all_doors.Closing3.Button_detection.Timer_LL.Set
            Init_procedure.Closing_all_doors.Closing3.Button_detection.Timer_LL.Set -> (junction 67711)
            (junction 67711) -> Init_procedure.Closing_all_doors.Closing3.Button_detection.Timer_LL.Counting [order 1] : [ET_LL<PT_LL]
            (junction 67711) -> (junction 67710) [order 2]
          state BUTTON_DOWN
            state Button_DOWN_1
              en:
              BUTTON_DOWN(2)=true;
              BUT_TEMP=1;
              LPD1=true;
              PUSHED=true;
              UPDATE=false;
              IN_LL=false; ET_LL=0;
            state First_but_1
              en:
              BUT_1=BUT_TEMP;
              FIRST_BUT=false;
            state Button_DOWN_2
              en:
              BUTTON_DOWN(3)=true;
              BUT_TEMP=2;
              LPD2=true;
              PUSHED=true;
              UPDATE=false;
              IN_LL=false; ET_LL=0;
            state First_but_2
              en:
              BUT_1=BUT_TEMP;
              FIRST_BUT=false;
            state Button_DOWN_3
              en:
              BUTTON_DOWN(4)=true;
              BUT_TEMP=3;
              LPD3=true;
              PUSHED=true;
              UPDATE=false;
              IN_LL=false; ET_LL=0;
            state First_but_3
              en:
              BUT_1=BUT_TEMP;
              FIRST_BUT=false;
            (default) -> (junction 67724)
            (junction 67724) -> Init_procedure.Closing_all_doors.Closing3.Button_detection.BUTTON_DOWN.Button_DOWN_1 [order 1] : [PD1]
            Init_procedure.Closing_all_doors.Closing3.Button_detection.BUTTON_DOWN.Button_DOWN_1 -> (junction 67725)
            (junction 67725) -> Init_procedure.Closing_all_doors.Closing3.Button_detection.BUTTON_DOWN.First_but_1 [order 1] : [FIRST_BUT && not(RPC1)]
            Init_procedure.Closing_all_doors.Closing3.Button_detection.BUTTON_DOWN.First_but_1 -> (junction 67726)
            (junction 67724) -> (junction 67727) [order 2]
            (junction 67725) -> (junction 67728) [order 2]
            (junction 67726) -> (junction 67729)
            (junction 67728) -> (junction 67727)
            (junction 67729) -> (junction 67728)
            (junction 67727) -> (junction 67730)
            (junction 67730) -> Init_procedure.Closing_all_doors.Closing3.Button_detection.BUTTON_DOWN.Button_DOWN_2 [order 1] : [PD2]
            Init_procedure.Closing_all_doors.Closing3.Button_detection.BUTTON_DOWN.Button_DOWN_2 -> (junction 67731)
            (junction 67731) -> Init_procedure.Closing_all_doors.Closing3.Button_detection.BUTTON_DOWN.First_but_2 [order 1] : [FIRST_BUT && not(RPC2)]
            Init_procedure.Closing_all_doors.Closing3.Button_detection.BUTTON_DOWN.First_but_2 -> (junction 67732)
            (junction 67730) -> (junction 67733) [order 2]
            (junction 67731) -> (junction 67734) [order 2]
            (junction 67732) -> (junction 67735)
            (junction 67734) -> (junction 67733)
            (junction 67735) -> (junction 67734)
            (junction 67733) -> (junction 67736)
            (junction 67736) -> Init_procedure.Closing_all_doors.Closing3.Button_detection.BUTTON_DOWN.Button_DOWN_3 [order 1] : [PD3]
            Init_procedure.Closing_all_doors.Closing3.Button_detection.BUTTON_DOWN.Button_DOWN_3 -> (junction 67737)
            (junction 67737) -> Init_procedure.Closing_all_doors.Closing3.Button_detection.BUTTON_DOWN.First_but_3 [order 1] : [FIRST_BUT && not(RPC3)]
            Init_procedure.Closing_all_doors.Closing3.Button_detection.BUTTON_DOWN.First_but_3 -> (junction 67738)
            (junction 67736) -> (junction 67739) [order 2]
            (junction 67737) -> (junction 67740) [order 2]
            (junction 67738) -> (junction 67741)
            (junction 67740) -> (junction 67739)
            (junction 67741) -> (junction 67740)
          state BUTTON_CAR
            state Button_CAR_0
              en:
              BUTTON_CAR(1)=true;
              BUT_TEMP=0;
              LPC0=true;
              PUSHED=true;
              UPDATE=false;
              IN_LL=false; ET_LL=0;
            state First_but_0
              en:
              BUT_1=BUT_TEMP;
              FIRST_BUT=false;
            state Button_CAR_1
              en:
              BUTTON_CAR(2)=true;
              BUT_TEMP=1;
              LPC1=true;
              PUSHED=true;
              UPDATE=false;
              IN_LL=false; ET_LL=0;
            state First_but_1
              en:
              BUT_1=BUT_TEMP;
              FIRST_BUT=false;
            state Button_CAR_2
              en:
              BUTTON_CAR(3)=true;
              BUT_TEMP=2;
              LPC2=true;
              PUSHED=true;
              UPDATE=false;
              IN_LL=false; ET_LL=0;
            state First_but_2
              en:
              BUT_1=BUT_TEMP;
              FIRST_BUT=false;
            state Button_CAR_3
              en:
              BUTTON_CAR(4)=true;
              BUT_TEMP=3;
              LPC3=true;
              PUSHED=true;
              UPDATE=false;
              IN_LL=false; ET_LL=0;
            state First_but_3
              en:
              BUT_1=BUT_TEMP;
              FIRST_BUT=false;
            (default) -> (junction 67779)
            (junction 67779) -> Init_procedure.Closing_all_doors.Closing3.Button_detection.BUTTON_CAR.Button_CAR_0 [order 1] : [P0]
            Init_procedure.Closing_all_doors.Closing3.Button_detection.BUTTON_CAR.Button_CAR_0 -> (junction 67780)
            (junction 67780) -> Init_procedure.Closing_all_doors.Closing3.Button_detection.BUTTON_CAR.First_but_0 [order 1] : [FIRST_BUT && not(RPC0)]
            Init_procedure.Closing_all_doors.Closing3.Button_detection.BUTTON_CAR.First_but_0 -> (junction 67781)
            (junction 67779) -> (junction 67782) [order 2]
            (junction 67780) -> (junction 67783) [order 2]
            (junction 67781) -> (junction 67784)
            (junction 67783) -> (junction 67782)
            (junction 67784) -> (junction 67783)
            (junction 67782) -> (junction 67787)
            Init_procedure.Closing_all_doors.Closing3.Button_detection.BUTTON_CAR.Button_CAR_1 -> (junction 67785)
            (junction 67785) -> Init_procedure.Closing_all_doors.Closing3.Button_detection.BUTTON_CAR.First_but_1 [order 1] : [FIRST_BUT && not(RPC1)]
            Init_procedure.Closing_all_doors.Closing3.Button_detection.BUTTON_CAR.First_but_1 -> (junction 67786)
            (junction 67785) -> (junction 67789) [order 2]
            (junction 67786) -> (junction 67790)
            (junction 67787) -> Init_procedure.Closing_all_doors.Closing3.Button_detection.BUTTON_CAR.Button_CAR_1 [order 1] : [P1]
            (junction 67787) -> (junction 67788) [order 2]
            (junction 67789) -> (junction 67788)
            (junction 67790) -> (junction 67789)
            (junction 67788) -> (junction 67791)
            (junction 67791) -> Init_procedure.Closing_all_doors.Closing3.Button_detection.BUTTON_CAR.Button_CAR_2 [order 1] : [P2]
            Init_procedure.Closing_all_doors.Closing3.Button_detection.BUTTON_CAR.Button_CAR_2 -> (junction 67792)
            (junction 67792) -> Init_procedure.Closing_all_doors.Closing3.Button_detection.BUTTON_CAR.First_but_2 [order 1] : [FIRST_BUT && not(RPC2)]
            Init_procedure.Closing_all_doors.Closing3.Button_detection.BUTTON_CAR.First_but_2 -> (junction 67793)
            (junction 67791) -> (junction 67794) [order 2]
            (junction 67792) -> (junction 67795) [order 2]
            (junction 67793) -> (junction 67796)
            (junction 67795) -> (junction 67794)
            (junction 67796) -> (junction 67795)
            (junction 67794) -> (junction 67797)
            (junction 67797) -> Init_procedure.Closing_all_doors.Closing3.Button_detection.BUTTON_CAR.Button_CAR_3 [order 1] : [P3]
            Init_procedure.Closing_all_doors.Closing3.Button_detection.BUTTON_CAR.Button_CAR_3 -> (junction 67798)
            (junction 67798) -> Init_procedure.Closing_all_doors.Closing3.Button_detection.BUTTON_CAR.First_but_3 [order 1] : [FIRST_BUT && not(RPC3)]
            Init_procedure.Closing_all_doors.Closing3.Button_detection.BUTTON_CAR.First_but_3 -> (junction 67799)
            (junction 67797) -> (junction 67800) [order 2]
            (junction 67798) -> (junction 67801) [order 2]
            (junction 67799) -> (junction 67802)
            (junction 67801) -> (junction 67800)
            (junction 67802) -> (junction 67801)
          state BUTTON_UP
            state Button_UP_0
              en:
              BUTTON_UP(1)=true;
              BUT_TEMP=0;
              LPS0=true;
              PUSHED=true;
              UPDATE=false;
              IN_LL=false; ET_LL=0;
            state First_but_0
              en:
              BUT_1=BUT_TEMP;
              FIRST_BUT=false;
            state Button_UP_1
              en:
              BUTTON_UP(2)=true;
              BUT_TEMP=1;
              LPS1=true;
              PUSHED=true;
              UPDATE=false;
              IN_LL=false; ET_LL=0;
            state First_but_1
              en:
              BUT_1=BUT_TEMP;
              FIRST_BUT=false;
            state Button_UP_2
              en:
              BUTTON_UP(3)=true;
              BUT_TEMP=2;
              LPS2=true;
              PUSHED=true;
              UPDATE=false;
              IN_LL=false; ET_LL=0;
            state First_but_2
              en:
              BUT_1=BUT_TEMP;
              FIRST_BUT=false;
            (junction 67852) -> Init_procedure.Closing_all_doors.Closing3.Button_detection.BUTTON_UP.Button_UP_0 [order 1] : [PS0]
            Init_procedure.Closing_all_doors.Closing3.Button_detection.BUTTON_UP.Button_UP_0 -> (junction 67853)
            (junction 67853) -> Init_procedure.Closing_all_doors.Closing3.Button_detection.BUTTON_UP.First_but_0 [order 1] : [FIRST_BUT && not(RPC0)]
            Init_procedure.Closing_all_doors.Closing3.Button_detection.BUTTON_UP.First_but_0 -> (junction 67854)
            (default) -> (junction 67852)
            (junction 67852) -> (junction 67857) [order 2]
            (junction 67853) -> (junction 67855) [order 2]
            (junction 67854) -> (junction 67856)
            (junction 67856) -> (junction 67855)
            (junction 67855) -> (junction 67857)
            (junction 67857) -> (junction 67858)
            (junction 67858) -> Init_procedure.Closing_all_doors.Closing3.Button_detection.BUTTON_UP.Button_UP_1 [order 1] : [PS1]
            Init_procedure.Closing_all_doors.Closing3.Button_detection.BUTTON_UP.Button_UP_1 -> (junction 67859)
            (junction 67859) -> Init_procedure.Closing_all_doors.Closing3.Button_detection.BUTTON_UP.First_but_1 [order 1] : [FIRST_BUT && not(RPC1)]
            Init_procedure.Closing_all_doors.Closing3.Button_detection.BUTTON_UP.First_but_1 -> (junction 67860)
            (junction 67858) -> (junction 67861) [order 2]
            (junction 67859) -> (junction 67862) [order 2]
            (junction 67860) -> (junction 67863)
            (junction 67862) -> (junction 67861)
            (junction 67863) -> (junction 67862)
            (junction 67861) -> (junction 67865)
            Init_procedure.Closing_all_doors.Closing3.Button_detection.BUTTON_UP.First_but_2 -> (junction 67864)
            (junction 67864) -> (junction 67869)
            (junction 67865) -> Init_procedure.Closing_all_doors.Closing3.Button_detection.BUTTON_UP.Button_UP_2 [order 1] : [PS2]
            Init_procedure.Closing_all_doors.Closing3.Button_detection.BUTTON_UP.Button_UP_2 -> (junction 67866)
            (junction 67866) -> Init_procedure.Closing_all_doors.Closing3.Button_detection.BUTTON_UP.First_but_2 [order 1] : [FIRST_BUT && not(RPC2)]
            (junction 67865) -> (junction 67867) [order 2]
            (junction 67866) -> (junction 67868) [order 2]
            (junction 67868) -> (junction 67867)
            (junction 67869) -> (junction 67868)
          state Max_Min_assignment
            state Min_but
              en:
              BUTTON=MIN_BUT;
            state Max_but
              en:
              BUTTON=MAX_BUT;
            state First_but
              en:
              BUTTON=BUT_1;
            state Max_but1
              en:
              MAX_BUT=2;
            state Max_but2
              en:
              MAX_BUT=1;
            state Max_but3
              en:
              MAX_BUT=0;
            state Min_but1
              en:
              MIN_BUT=1;
            state Min_but2
              en:
              MIN_BUT=2;
            state Min_but3
              en:
              MIN_BUT=3;
            state MAX
              en:
              MAX_BUT=BUT_TEMP;
            state MIN
              en:
              MIN_BUT=BUT_TEMP;
            state Updating_button_0
              en:
              BUTTON=MAX_BUT;
            state Updating_button_1
              en:
              BUTTON=MIN_BUT;
            (junction 67907) -> Init_procedure.Closing_all_doors.Closing3.Button_detection.Max_Min_assignment.Min_but [order 1] : [(MAX_BUT-FLOOR)>(FLOOR-MIN_BUT)]
            Init_procedure.Closing_all_doors.Closing3.Button_detection.Max_Min_assignment.Min_but -> (junction 67908)
            (junction 67909) -> (junction 67907) [order 1] : [not(FLAG_STOP) && MOTION==2 && FLAG==3]
            (default) -> (junction 67909)
            (junction 67907) -> (junction 67910) [order 2]
            (junction 67908) -> (junction 67911)
            (junction 67909) -> (junction 67912) [order 2]
            (junction 67910) -> Init_procedure.Closing_all_doors.Closing3.Button_detection.Max_Min_assignment.Max_but [order 1] : [(MAX_BUT-FLOOR)<(FLOOR-MIN_BUT)]
            Init_procedure.Closing_all_doors.Closing3.Button_detection.Max_Min_assignment.Max_but -> (junction 67911)
            (junction 67910) -> Init_procedure.Closing_all_doors.Closing3.Button_detection.Max_Min_assignment.First_but [order 2]
            (junction 67911) -> (junction 67914)
            Init_procedure.Closing_all_doors.Closing3.Button_detection.Max_Min_assignment.First_but -> (junction 67913)
            (junction 67913) -> (junction 67912)
            (junction 67914) -> (junction 67913)
            (junction 67912) -> (junction 67915)
            (junction 67916) -> (junction 67917) [order 1] : [MOTION==0]
                | {MOTION=1;
                | UPDATE=true;}
            (junction 67917) -> Init_procedure.Closing_all_doors.Closing3.Button_detection.Max_Min_assignment.Max_but1 [order 1] : [BUTTON_UP(2)]
            Init_procedure.Closing_all_doors.Closing3.Button_detection.Max_Min_assignment.Max_but1 -> (junction 67918)
            (junction 67915) -> (junction 67916) [order 1] : [BUTTON==FLOOR && EXTEND]
                | {EXTEND=false;}
            (junction 67915) -> (junction 67929) [order 2]
            (junction 67916) -> (junction 67921) [order 2]
            (junction 67917) -> (junction 67919) [order 2]
            (junction 67918) -> (junction 67920)
            (junction 67919) -> Init_procedure.Closing_all_doors.Closing3.Button_detection.Max_Min_assignment.Max_but2 [order 1] : [BUTTON_UP(1)]
            Init_procedure.Closing_all_doors.Closing3.Button_detection.Max_Min_assignment.Max_but2 -> (junction 67920)
            (junction 67919) -> Init_procedure.Closing_all_doors.Closing3.Button_detection.Max_Min_assignment.Max_but3 [order 2]
            (junction 67920) -> (junction 67923)
            Init_procedure.Closing_all_doors.Closing3.Button_detection.Max_Min_assignment.Max_but3 -> (junction 67922)
            (junction 67922) -> (junction 67921)
            (junction 67923) -> (junction 67922)
            (junction 67921) -> (junction 67924)
            (junction 67924) -> (junction 67925) [order 1] : [MOTION==1]
                | {MOTION=0;
                | UPDATE=true;}
            (junction 67925) -> Init_procedure.Closing_all_doors.Closing3.Button_detection.Max_Min_assignment.Min_but1 [order 1] : [BUTTON_DOWN(1)]
            Init_procedure.Closing_all_doors.Closing3.Button_detection.Max_Min_assignment.Min_but1 -> (junction 67926)
            (junction 67924) -> (junction 67930) [order 2]
            (junction 67925) -> (junction 67927) [order 2]
            (junction 67926) -> (junction 67928)
            (junction 67927) -> Init_procedure.Closing_all_doors.Closing3.Button_detection.Max_Min_assignment.Min_but2 [order 1] : [BUTTON_DOWN(2)]
            Init_procedure.Closing_all_doors.Closing3.Button_detection.Max_Min_assignment.Min_but2 -> (junction 67928)
            (junction 67927) -> Init_procedure.Closing_all_doors.Closing3.Button_detection.Max_Min_assignment.Min_but3 [order 2]
            (junction 67928) -> (junction 67932)
            Init_procedure.Closing_all_doors.Closing3.Button_detection.Max_Min_assignment.Min_but3 -> (junction 67931)
            (junction 67930) -> (junction 67929)
            (junction 67931) -> (junction 67930)
            (junction 67932) -> (junction 67931)
            (junction 67929) -> (junction 67934)
            Init_procedure.Closing_all_doors.Closing3.Button_detection.Max_Min_assignment.MAX -> (junction 67933)
            (junction 67934) -> (junction 67935) [order 1] : [PUSHED]
            (junction 67935) -> (junction 67936) [order 1] : [not(BUT_TEMP==FLOOR) || not(MOTION==2)]
            (junction 67936) -> Init_procedure.Closing_all_doors.Closing3.Button_detection.Max_Min_assignment.MAX [order 1] : [MAX_BUT<BUT_TEMP && not(UPDATE)]
            (junction 67933) -> (junction 67938)
            (junction 67934) -> (junction 67948) [order 2]
            (junction 67935) -> (junction 67941) [order 2]
            (junction 67936) -> (junction 67937) [order 2]
            (junction 67938) -> (junction 67937)
            (junction 67937) -> (junction 67939)
            (junction 67939) -> Init_procedure.Closing_all_doors.Closing3.Button_detection.Max_Min_assignment.MIN [order 1] : [MIN_BUT>BUT_TEMP && not(UPDATE)]
            Init_procedure.Closing_all_doors.Closing3.Button_detection.Max_Min_assignment.MIN -> (junction 67940)
            (junction 67939) -> (junction 67942) [order 2]
            (junction 67940) -> (junction 67943)
            (junction 67942) -> (junction 67941)
            (junction 67943) -> (junction 67942)
            (junction 67941) -> (junction 67944)
            (junction 67944) -> Init_procedure.Closing_all_doors.Closing3.Button_detection.Max_Min_assignment.Updating_button_0 [order 1] : [MOTION==0]
            Init_procedure.Closing_all_doors.Closing3.Button_detection.Max_Min_assignment.Updating_button_0 -> (junction 67945)
            (junction 67944) -> (junction 67946) [order 2]
            (junction 67945) -> (junction 67947)
            (junction 67946) -> Init_procedure.Closing_all_doors.Closing3.Button_detection.Max_Min_assignment.Updating_button_1 [order 1] : [MOTION==1]
            Init_procedure.Closing_all_doors.Closing3.Button_detection.Max_Min_assignment.Updating_button_1 -> (junction 67947)
            (junction 67946) -> (junction 67949) [order 2]
            (junction 67947) -> (junction 67950)
            (junction 67949) -> (junction 67948)
            (junction 67950) -> (junction 67949)
          state GoTo_PositionControl
            en:
            BUTTON=BUT_TEMP;
            FLAG=2;
          state Emergency
            en:
            FLAG_EMG=true;
            FLAG=4;
          state Timer_EME
            state Set_tmr
              en:
              Q_EME=true;
            state Counting
              en:
              ET_EME= ET_EME + 1;
              Q_EME=false;
            state Set
              en:
              IN_EME=true;
              PT_EME=3;
            (junction 68040) -> Init_procedure.Closing_all_doors.Closing3.Button_detection.Timer_EME.Set_tmr [order 1] : [ET_EME==PT_EME]
            Init_procedure.Closing_all_doors.Closing3.Button_detection.Timer_EME.Set_tmr -> (junction 68041)
            Init_procedure.Closing_all_doors.Closing3.Button_detection.Timer_EME.Counting -> (junction 68040)
            (junction 68040) -> (junction 68041) [order 2]
            (default) -> Init_procedure.Closing_all_doors.Closing3.Button_detection.Timer_EME.Set
            Init_procedure.Closing_all_doors.Closing3.Button_detection.Timer_EME.Set -> (junction 68042)
            (junction 68042) -> Init_procedure.Closing_all_doors.Closing3.Button_detection.Timer_EME.Counting [order 1] : [ET_EME<PT_EME]
            (junction 68042) -> (junction 68041) [order 2]
          state Not_Emergency
            en:
            IN_EME=false;
            ET_EME=0;
          state SwitchingOFF_LEDs
            en:
            LPD3=false;
            LPD2=false;
            LPS2=false;
            LPD1=false;
            LPS1=false;
            LPS0=false;
          (default) -> (junction 67641)
          (junction 67641) -> (junction 67642) [order 1] : [FLAG==1 && not(PUSHED)]
              | {BUTTON=FLOOR;
              | BUT_TEMP=BUTTON;
              | BUT_1=FLOOR;}
          (junction 67642) -> Init_procedure.Closing_all_doors.Closing3.Button_detection.Timer_LL [order 1] : [not(FLAG_STOP)]
          Init_procedure.Closing_all_doors.Closing3.Button_detection.Save_energy -> (junction 67643)
          Init_procedure.Closing_all_doors.Closing3.Button_detection.Timer_LL -> Init_procedure.Closing_all_doors.Closing3.Button_detection.Save_energy
          (junction 67642) -> (junction 67645) [order 2]
          (junction 67641) -> (junction 67644) [order 2]
          (junction 67643) -> (junction 67646)
          (junction 67645) -> (junction 67644)
          (junction 67646) -> (junction 67645)
          (junction 67644) -> Init_procedure.Closing_all_doors.Closing3.Button_detection.BUTTON_CAR
          Init_procedure.Closing_all_doors.Closing3.Button_detection.BUTTON_UP -> Init_procedure.Closing_all_doors.Closing3.Button_detection.BUTTON_DOWN
          Init_procedure.Closing_all_doors.Closing3.Button_detection.BUTTON_DOWN -> Init_procedure.Closing_all_doors.Closing3.Button_detection.Max_Min_assignment
          Init_procedure.Closing_all_doors.Closing3.Button_detection.Max_Min_assignment -> (junction 67647)
          Init_procedure.Closing_all_doors.Closing3.Button_detection.BUTTON_CAR -> Init_procedure.Closing_all_doors.Closing3.Button_detection.BUTTON_UP
          (junction 67647) -> (junction 67649)
          (junction 67649) -> (junction 67648)
          (junction 67648) -> (junction 67651)
          Init_procedure.Closing_all_doors.Closing3.Button_detection.GoTo_PositionControl -> (junction 67650)
          (junction 67651) -> (junction 67652) [order 1] : [FLAG==1]
          (junction 67652) -> Init_procedure.Closing_all_doors.Closing3.Button_detection.GoTo_PositionControl [order 1] : [PUSHED]
          (junction 67650) -> (junction 67654)
          (junction 67651) -> (junction 67662) [order 2]
          (junction 67652) -> (junction 67653) [order 2]
          (junction 67654) -> (junction 67653)
          (junction 67653) -> (junction 67656)
          Init_procedure.Closing_all_doors.Closing3.Button_detection.Emergency -> (junction 67655)
          (junction 67656) -> Init_procedure.Closing_all_doors.Closing3.Button_detection.Timer_EME [order 1] : [STOP]
              | {IN_LL=false; ET_LL=0;FLAG=1;}
          Init_procedure.Closing_all_doors.Closing3.Button_detection.Timer_EME -> (junction 67657)
          (junction 67657) -> Init_procedure.Closing_all_doors.Closing3.Button_detection.Emergency [order 1] : [Q_EME]
          (junction 67655) -> (junction 67659)
          (junction 67656) -> Init_procedure.Closing_all_doors.Closing3.Button_detection.Not_Emergency [order 2]
          (junction 67657) -> (junction 67658) [order 2]
          (junction 67659) -> (junction 67658)
          (junction 67658) -> (junction 67661)
          Init_procedure.Closing_all_doors.Closing3.Button_detection.Not_Emergency -> (junction 67661)
          Init_procedure.Closing_all_doors.Closing3.Button_detection.SwitchingOFF_LEDs -> (junction 67660)
          (junction 67661) -> Init_procedure.Closing_all_doors.Closing3.Button_detection.SwitchingOFF_LEDs [order 1] : [FLAG_STOP && FLAG==2]
          (junction 67660) -> (junction 67664)
          (junction 67661) -> (junction 67663) [order 2]
          (junction 67663) -> (junction 67662)
          (junction 67664) -> (junction 67663)
        state Extending
          en:
          EXTEND=true;
        state Stop_Closing
          en:
          CP2=false;
          FLAG_OD=false;
          OBS=false;
          ET_cl=0;
          IN_cl=false;
        state GoTo_PositionControl
          en: FLAG=2;
        state GoTo_BUttonDetection
          en:
          MOTION=2;
          MAX_BUT=0;
          MIN_BUT=3;
          PUSHED=false;
          FIRST_BUT=true;
          FLAG=1;
          UPDATE=false;
        state Closing1
          en:CP2=true;
        state Stop_Closing1
          en:CP2=false;
        Init_procedure.Closing_all_doors.Closing3.Reset -> Init_procedure.Closing_all_doors.Closing3.Timer_close
        (default) -> (junction 67552)
        (junction 67552) -> Init_procedure.Closing_all_doors.Closing3.Reset [order 1] : [not(FLAG==0) && not(FLAG==4)]
        Init_procedure.Closing_all_doors.Closing3.Timer_close -> (junction 67553)
        (junction 67553) -> Init_procedure.Closing_all_doors.Closing3.Closing [order 1] : [not(PC2)]
        Init_procedure.Closing_all_doors.Closing3.Button_detection -> (junction 67554)
        Init_procedure.Closing_all_doors.Closing3.Closing -> Init_procedure.Closing_all_doors.Closing3.Button_detection
        (junction 67552) -> (junction 67562) [order 2]
        (junction 67553) -> (junction 67555) [order 2]
        (junction 67554) -> (junction 67560)
        (junction 67555) -> Init_procedure.Closing_all_doors.Closing3.Extending [order 1] : [BUTTON==FLOOR]
        (junction 67555) -> (junction 67557) [order 2]
        Init_procedure.Closing_all_doors.Closing3.Extending -> (junction 67556)
        (junction 67556) -> (junction 67557)
        (junction 67557) -> Init_procedure.Closing_all_doors.Closing3.Stop_Closing
        Init_procedure.Closing_all_doors.Closing3.Stop_Closing -> (junction 67558)
        (junction 67558) -> Init_procedure.Closing_all_doors.Closing3.GoTo_PositionControl [order 2]
        (junction 67558) -> Init_procedure.Closing_all_doors.Closing3.GoTo_BUttonDetection [order 1] : [not(BUTTON_CAR(1) || BUTTON_CAR(2) || BUTTON_CAR(3) || BUTTON_CAR(4) || BUTTON_UP(1) || BUTTON_UP(2) || BUTTON_UP(3) || BUTTON_DOWN(2) || BUTTON_DOWN(3) || BUTTON_DOWN(4))]
        Init_procedure.Closing_all_doors.Closing3.GoTo_PositionControl -> (junction 67559)
        Init_procedure.Closing_all_doors.Closing3.GoTo_BUttonDetection -> (junction 67559)
        (junction 67559) -> (junction 67560)
        (junction 67560) -> (junction 67561)
        (junction 67561) -> (junction 67563)
        (junction 67562) -> Init_procedure.Closing_all_doors.Closing3.Closing1 [order 1] : [not(PC2)]
        Init_procedure.Closing_all_doors.Closing3.Closing1 -> (junction 67563)
        (junction 67562) -> Init_procedure.Closing_all_doors.Closing3.Stop_Closing1 [order 2]
        Init_procedure.Closing_all_doors.Closing3.Stop_Closing1 -> (junction 67563)
      Init_procedure.Closing_all_doors.Closing0 -> Init_procedure.Closing_all_doors.Closing1
      (default) -> Init_procedure.Closing_all_doors.Closing0
      Init_procedure.Closing_all_doors.Closing1 -> (junction 27074)
      (junction 27074) -> (junction 27073)
      (junction 27073) -> Init_procedure.Closing_all_doors.Closing2
      Init_procedure.Closing_all_doors.Closing2 -> Init_procedure.Closing_all_doors.Closing3
    state Replacing
      en:
      SCENDI=true;
    state Replaced
      en:
      SCENDI=false;
    state End_init
      en:
      FLAG=1;
      LPS0=false;LPS1=false;
      LPS2=false;LPD2=false;
      LPD3=false;LPD1=false;
      BUT_TEMP=FLOOR;
    (default) -> BLK_Init
    BLK_Init -> Closing_all_doors
    Closing_all_doors -> (junction 27051)
    (junction 27051) -> (junction 27053)
    (junction 27053) -> (junction 27064)
    (junction 27064) -> Init_procedure.Replacing [order 1] : [not(RPC0) && not(RPC1) && not(RPC2) && not(RPC3)]
    Init_procedure.Replacing -> (junction 27057)
    (junction 27064) -> Init_procedure.Replaced [order 2]
    Init_procedure.Replaced -> (junction 27057)
    (junction 27057) -> (junction 27060)
    (junction 27060) -> (junction 27062)
    (junction 27062) -> (junction 27066)
    (junction 27066) -> End_init [order 1] : [(RPC0 || RPC1 || RPC2 || RPC3) && (PC0 && PC1 && PC2 && PC3)]
    (junction 27066) -> (junction 27068) [order 2]
    End_init -> (junction 27068)
  state Blackout
    state OFF
      en:
      FLAG_BO=true;
      AP0=false;
      AP1=false;
      AP2=false;
      AP3=false;
      CP0=false;
      CP1=false;
      CP2=false;
      CP3=false;
      SALI=false;
      SCENDI=false;
      LL=false;
      LPC0=false;
      LPC1=false;
      LPC2=false;
      LPC3=false;
      LPS0=false;
      LPS1=false;
      LPD1=false;
      LPS2=false;
      LPD2=false;
      LPD3=false;
      BUTTON_CAR(1)=false;
      BUTTON_CAR(2)=false;
      BUTTON_CAR(3)=false;
      BUTTON_CAR(4)=false;
      BUTTON_UP(1)=false;
      BUTTON_UP(2)=false;
      BUTTON_UP(3)=false;
      BUTTON_UP(4)=false;
      BUTTON_DOWN(1)=false;
      BUTTON_DOWN(2)=false;
      BUTTON_DOWN(3)=false;
      BUTTON_DOWN(4)=false;
      FLAG=5;
      IN_LL=false; ET_LL=0;
    state ON
      en:
      LL=true;
    state Start_recovery
      en:
      FLAG_REC=true;
      FLAG=4;
    (junction 4492) -> OFF [order 1] : [BO && not(FLAG_BO) && not(RECOVERY)]
    (default) -> (junction 4492)
    OFF -> (junction 58088)
    (junction 4492) -> (junction 26907) [order 2]
    (junction 58088) -> (junction 58089)
    (junction 26907) -> ON [order 1] : [not(BO) && not(RECOVERY)]
    ON -> (junction 58089)
    (junction 26907) -> (junction 58086) [order 2]
    (junction 58089) -> (junction 26909)
    (junction 26909) -> (junction 58086)
    (junction 58086) -> (junction 58094)
    (junction 58094) -> Start_recovery [order 1] : [RECOVERY]
    Start_recovery -> (junction 58096)
    (junction 58094) -> (junction 26913) [order 2]
    (junction 58096) -> (junction 58097)
    (junction 26913) -> (junction 58097)
  state Fire_detection
    state Firing
      en:
      FLAG=4;
      FLAG_EMG=true;
      SALI=false;
      BUTTON_CAR(1)=false;
      BUTTON_CAR(2)=false;
      BUTTON_CAR(3)=false;
      BUTTON_CAR(4)=false;
      BUTTON_UP(1)=false;
      BUTTON_UP(2)=false;
      BUTTON_UP(3)=false;
      BUTTON_UP(4)=false;
      BUTTON_DOWN(1)=false;
      BUTTON_DOWN(2)=false;
      BUTTON_DOWN(3)=false;
      BUTTON_DOWN(4)=false;
    state NOT_fire
    (junction 26902) -> Firing [order 1] : [FIRE]
    (default) -> (junction 26902)
    Firing -> (junction 26903)
    (junction 26902) -> (junction 58104) [order 2]
    (junction 26903) -> (junction 58105)
    (junction 58104) -> NOT_fire
    NOT_fire -> (junction 58105)
  state Floor_detection
    state F0
      en:
      FLOOR=0;
      LPC0=true;
    state NOT_F0
      en:
      LPC0=false;
    state F1
      en:
      FLOOR=1;
      LPC1=true;
    state NOT_F1
      en:
      LPC1=false;
    state F2
      en:
      FLOOR=2;
      LPC2=true;
    state NOT_F2
      en:
      LPC2=false;
    state F3
      en:
      FLOOR=3;
      LPC3=true;
    state NOT_F3
      en:
      LPC3=false;
    (default) -> (junction 11229)
    (junction 11229) -> F0 [order 1] : [RPC0]
    F0 -> (junction 27006)
    (junction 11229) -> (junction 27004) [order 2]
    (junction 27006) -> (junction 27009)
    (junction 27004) -> NOT_F0 [order 1] : [not(BUTTON_CAR(1))]
    NOT_F0 -> (junction 27009)
    (junction 27009) -> (junction 27008)
    (junction 27004) -> (junction 27008) [order 2]
    (junction 27008) -> F1 [order 1] : [RPC1]
    (junction 27008) -> (junction 27014) [order 2]
    F1 -> (junction 27018)
    (junction 27018) -> (junction 27020)
    NOT_F1 -> (junction 27020)
    (junction 27014) -> NOT_F1 [order 1] : [not(BUTTON_CAR(2))]
    (junction 27020) -> (junction 27022)
    (junction 27014) -> (junction 27022) [order 2]
    (junction 27022) -> F2 [order 1] : [RPC2]
    (junction 27022) -> (junction 27030) [order 2]
    F2 -> (junction 27026)
    (junction 27026) -> (junction 27029)
    NOT_F2 -> (junction 27029)
    (junction 27030) -> NOT_F2 [order 1] : [not(BUTTON_CAR(3))]
    (junction 27029) -> (junction 27032)
    (junction 27030) -> (junction 27032) [order 2]
    (junction 27032) -> F3 [order 1] : [RPC3]
    (junction 27032) -> (junction 27034) [order 2]
    F3 -> (junction 27045)
    (junction 27045) -> (junction 27048)
    (junction 27034) -> NOT_F3 [order 1] : [not(BUTTON_CAR(4))]
    NOT_F3 -> (junction 27048)
    (junction 27048) -> (junction 27049)
    (junction 27034) -> (junction 27049) [order 2]
  state Button_detection
    state Save_energy
      en:
      LL=not(Q_LL);
    state Timer_LL
      state Set_tmr
        en:
        Q_LL=true;
      state Counting
        en:
        ET_LL= ET_LL + 1;
        Q_LL=false;
      state Set
        en:
        IN_LL=true;
        PT_LL=10;
      (junction 29079) -> Button_detection.Timer_LL.Set_tmr [order 1] : [ET_LL==PT_LL]
      Button_detection.Timer_LL.Set_tmr -> (junction 29080)
      Button_detection.Timer_LL.Counting -> (junction 29079)
      (junction 29079) -> (junction 29080) [order 2]
      (default) -> Button_detection.Timer_LL.Set
      Button_detection.Timer_LL.Set -> (junction 29081)
      (junction 29081) -> Button_detection.Timer_LL.Counting [order 1] : [ET_LL<PT_LL]
      (junction 29081) -> (junction 29080) [order 2]
    state BUTTON_DOWN
      state Button_DOWN_1
        en:
        BUTTON_DOWN(2)=true;
        BUT_TEMP=1;
        LPD1=true;
        PUSHED=true;
        UPDATE=false;
        IN_LL=false; ET_LL=0;
      state First_but_1
        en:
        BUT_1=BUT_TEMP;
        FIRST_BUT=false;
      state Button_DOWN_2
        en:
        BUTTON_DOWN(3)=true;
        BUT_TEMP=2;
        LPD2=true;
        PUSHED=true;
        UPDATE=false;
        IN_LL=false; ET_LL=0;
      state First_but_2
        en:
        BUT_1=BUT_TEMP;
        FIRST_BUT=false;
      state Button_DOWN_3
        en:
        BUTTON_DOWN(4)=true;
        BUT_TEMP=3;
        LPD3=true;
        PUSHED=true;
        UPDATE=false;
        IN_LL=false; ET_LL=0;
      state First_but_3
        en:
        BUT_1=BUT_TEMP;
        FIRST_BUT=false;
      (default) -> (junction 29094)
      (junction 29094) -> Button_detection.BUTTON_DOWN.Button_DOWN_1 [order 1] : [PD1]
      Button_detection.BUTTON_DOWN.Button_DOWN_1 -> (junction 29095)
      (junction 29095) -> Button_detection.BUTTON_DOWN.First_but_1 [order 1] : [FIRST_BUT && not(RPC1)]
      Button_detection.BUTTON_DOWN.First_but_1 -> (junction 29096)
      (junction 29094) -> (junction 29097) [order 2]
      (junction 29095) -> (junction 29098) [order 2]
      (junction 29096) -> (junction 29099)
      (junction 29098) -> (junction 29097)
      (junction 29099) -> (junction 29098)
      (junction 29097) -> (junction 29100)
      (junction 29100) -> Button_detection.BUTTON_DOWN.Button_DOWN_2 [order 1] : [PD2]
      Button_detection.BUTTON_DOWN.Button_DOWN_2 -> (junction 29101)
      (junction 29101) -> Button_detection.BUTTON_DOWN.First_but_2 [order 1] : [FIRST_BUT && not(RPC2)]
      Button_detection.BUTTON_DOWN.First_but_2 -> (junction 29102)
      (junction 29100) -> (junction 29103) [order 2]
      (junction 29101) -> (junction 29104) [order 2]
      (junction 29102) -> (junction 29105)
      (junction 29104) -> (junction 29103)
      (junction 29105) -> (junction 29104)
      (junction 29103) -> (junction 29106)
      (junction 29106) -> Button_detection.BUTTON_DOWN.Button_DOWN_3 [order 1] : [PD3]
      Button_detection.BUTTON_DOWN.Button_DOWN_3 -> (junction 29107)
      (junction 29107) -> Button_detection.BUTTON_DOWN.First_but_3 [order 1] : [FIRST_BUT && not(RPC3)]
      Button_detection.BUTTON_DOWN.First_but_3 -> (junction 29108)
      (junction 29106) -> (junction 29111) [order 2]
      (junction 29107) -> (junction 29109) [order 2]
      (junction 29108) -> (junction 29110)
      (junction 29109) -> (junction 29111)
      (junction 29110) -> (junction 29109)
    state BUTTON_CAR
      state Button_CAR_0
        en:
        BUTTON_CAR(1)=true;
        BUT_TEMP=0;
        LPC0=true;
        PUSHED=true;
        UPDATE=false;
        IN_LL=false; ET_LL=0;
      state First_but_0
        en:
        BUT_1=BUT_TEMP;
        FIRST_BUT=false;
      state Button_CAR_1
        en:
        BUTTON_CAR(2)=true;
        BUT_TEMP=1;
        LPC1=true;
        PUSHED=true;
        UPDATE=false;
        IN_LL=false; ET_LL=0;
      state First_but_1
        en:
        BUT_1=BUT_TEMP;
        FIRST_BUT=false;
      state Button_CAR_2
        en:
        BUTTON_CAR(3)=true;
        BUT_TEMP=2;
        LPC2=true;
        PUSHED=true;
        UPDATE=false;
        IN_LL=false; ET_LL=0;
      state First_but_2
        en:
        BUT_1=BUT_TEMP;
        FIRST_BUT=false;
      state Button_CAR_3
        en:
        BUTTON_CAR(4)=true;
        BUT_TEMP=3;
        LPC3=true;
        PUSHED=true;
        UPDATE=false;
        IN_LL=false; ET_LL=0;
      state First_but_3
        en:
        BUT_1=BUT_TEMP;
        FIRST_BUT=false;
      (default) -> (junction 29149)
      (junction 29149) -> Button_detection.BUTTON_CAR.Button_CAR_0 [order 1] : [P0]
      Button_detection.BUTTON_CAR.Button_CAR_0 -> (junction 29150)
      (junction 29150) -> Button_detection.BUTTON_CAR.First_but_0 [order 1] : [FIRST_BUT && not(RPC0)]
      Button_detection.BUTTON_CAR.First_but_0 -> (junction 29151)
      (junction 29149) -> (junction 29152) [order 2]
      (junction 29150) -> (junction 29153) [order 2]
      (junction 29151) -> (junction 29154)
      (junction 29153) -> (junction 29152)
      (junction 29154) -> (junction 29153)
      (junction 29152) -> (junction 29157)
      Button_detection.BUTTON_CAR.Button_CAR_1 -> (junction 29156)
      (junction 29156) -> Button_detection.BUTTON_CAR.First_but_1 [order 1] : [FIRST_BUT && not(RPC1)]
      Button_detection.BUTTON_CAR.First_but_1 -> (junction 29155)
      (junction 29156) -> (junction 29159) [order 2]
      (junction 29155) -> (junction 29160)
      (junction 29157) -> Button_detection.BUTTON_CAR.Button_CAR_1 [order 1] : [P1]
      (junction 29157) -> (junction 29158) [order 2]
      (junction 29159) -> (junction 29158)
      (junction 29160) -> (junction 29159)
      (junction 29158) -> (junction 29161)
      (junction 29161) -> Button_detection.BUTTON_CAR.Button_CAR_2 [order 1] : [P2]
      Button_detection.BUTTON_CAR.Button_CAR_2 -> (junction 29162)
      (junction 29162) -> Button_detection.BUTTON_CAR.First_but_2 [order 1] : [FIRST_BUT && not(RPC2)]
      Button_detection.BUTTON_CAR.First_but_2 -> (junction 29163)
      (junction 29161) -> (junction 29164) [order 2]
      (junction 29162) -> (junction 29165) [order 2]
      (junction 29163) -> (junction 29166)
      (junction 29165) -> (junction 29164)
      (junction 29166) -> (junction 29165)
      (junction 29164) -> (junction 29167)
      (junction 29167) -> Button_detection.BUTTON_CAR.Button_CAR_3 [order 1] : [P3]
      Button_detection.BUTTON_CAR.Button_CAR_3 -> (junction 29168)
      (junction 29168) -> Button_detection.BUTTON_CAR.First_but_3 [order 1] : [FIRST_BUT && not(RPC3)]
      Button_detection.BUTTON_CAR.First_but_3 -> (junction 29169)
      (junction 29167) -> (junction 29170) [order 2]
      (junction 29168) -> (junction 29171) [order 2]
      (junction 29169) -> (junction 29172)
      (junction 29171) -> (junction 29170)
      (junction 29172) -> (junction 29171)
    state BUTTON_UP
      state Button_UP_0
        en:
        BUTTON_UP(1)=true;
        BUT_TEMP=0;
        LPS0=true;
        PUSHED=true;
        UPDATE=false;
        IN_LL=false; ET_LL=0;
      state First_but_0
        en:
        BUT_1=BUT_TEMP;
        FIRST_BUT=false;
      state Button_UP_1
        en:
        BUTTON_UP(2)=true;
        BUT_TEMP=1;
        LPS1=true;
        PUSHED=true;
        UPDATE=false;
        IN_LL=false; ET_LL=0;
      state First_but_1
        en:
        BUT_1=BUT_TEMP;
        FIRST_BUT=false;
      state Button_UP_2
        en:
        BUTTON_UP(3)=true;
        BUT_TEMP=2;
        LPS2=true;
        PUSHED=true;
        UPDATE=false;
        IN_LL=false; ET_LL=0;
      state First_but_2
        en:
        BUT_1=BUT_TEMP;
        FIRST_BUT=false;
      (junction 29222) -> Button_detection.BUTTON_UP.Button_UP_0 [order 1] : [PS0]
      Button_detection.BUTTON_UP.Button_UP_0 -> (junction 29223)
      (junction 29223) -> Button_detection.BUTTON_UP.First_but_0 [order 1] : [FIRST_BUT && not(RPC0)]
      Button_detection.BUTTON_UP.First_but_0 -> (junction 29224)
      (default) -> (junction 29222)
      (junction 29222) -> (junction 29227) [order 2]
      (junction 29223) -> (junction 29225) [order 2]
      (junction 29224) -> (junction 29226)
      (junction 29226) -> (junction 29225)
      (junction 29225) -> (junction 29227)
      (junction 29227) -> (junction 29228)
      (junction 29228) -> Button_detection.BUTTON_UP.Button_UP_1 [order 1] : [PS1]
      Button_detection.BUTTON_UP.Button_UP_1 -> (junction 29229)
      (junction 29229) -> Button_detection.BUTTON_UP.First_but_1 [order 1] : [FIRST_BUT && not(RPC1)]
      Button_detection.BUTTON_UP.First_but_1 -> (junction 29230)
      (junction 29228) -> (junction 29231) [order 2]
      (junction 29229) -> (junction 29232) [order 2]
      (junction 29230) -> (junction 29233)
      (junction 29232) -> (junction 29231)
      (junction 29233) -> (junction 29232)
      (junction 29231) -> (junction 29235)
      Button_detection.BUTTON_UP.First_but_2 -> (junction 29234)
      (junction 29234) -> (junction 29239)
      (junction 29235) -> Button_detection.BUTTON_UP.Button_UP_2 [order 1] : [PS2]
      Button_detection.BUTTON_UP.Button_UP_2 -> (junction 29236)
      (junction 29236) -> Button_detection.BUTTON_UP.First_but_2 [order 1] : [FIRST_BUT && not(RPC2)]
      (junction 29235) -> (junction 29237) [order 2]
      (junction 29236) -> (junction 29238) [order 2]
      (junction 29238) -> (junction 29237)
      (junction 29239) -> (junction 29238)
    state Max_Min_assignment
      state Min_but
        en:
        BUTTON=MIN_BUT;
      state Max_but
        en:
        BUTTON=MAX_BUT;
      state First_but
        en:
        BUTTON=BUT_1;
      state Max_but1
        en:
        MAX_BUT=2;
      state Max_but2
        en:
        MAX_BUT=1;
      state Max_but3
        en:
        MAX_BUT=0;
      state Min_but1
        en:
        MIN_BUT=1;
      state Min_but2
        en:
        MIN_BUT=2;
      state Min_but3
        en:
        MIN_BUT=3;
      state MAX
        en:
        MAX_BUT=BUT_TEMP;
      state MIN
        en:
        MIN_BUT=BUT_TEMP;
